simulink library "rappid_564xl_ec_toolbox"  (R2016b)
settings: Solver=FixedStepDiscrete  StartTime=0.0  StopTime=10.0  RelTol=1e-3  EnableMultiTasking=on
undefined symbols (not defined in the file or in its folder): CTU_unit, mem_AddrLW, mem_AddrUP, rappid_564xl_adc_input_support_rev2, rappid_564xl_can_support_rev2, read_mem_AddrLW, read_mem_AddrUP
(part 4 of 6)

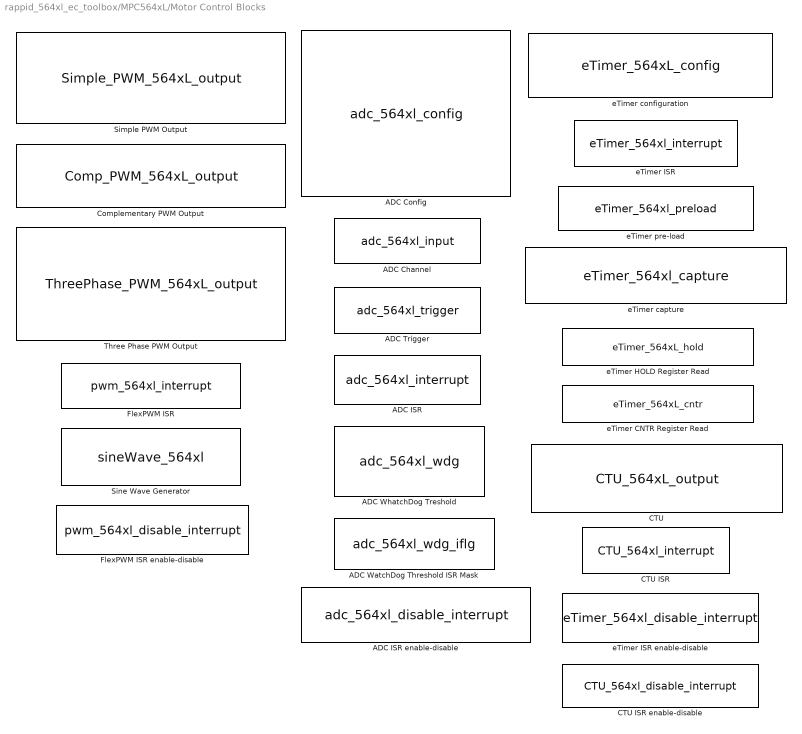
== system rappid_564xl_ec_toolbox/MPC564xL/Motor Control Blocks ==
  ADC Channel : S-Function  LoadFcn=rappid_564xl_adc_input_support_rev2(gcb)  FunctionName=adc_564xl_input  Parameters="adcChan, adc_unit, adc_mode, simulate,  interrupt, adc_presample"  SFunctionDeploymentMode=off  EnableBusSupport=off  mask(adc_564xl_input_block){adc_unit=1, adc_chan0=older, adc_chan0_v2=69 : PE5 : [44] : [T5] : AN8, adc_chan1=older, adc_chan1_v2=26 : PB10 : [53] : [R8] : AN12, simulate=off, interrupt=off, adc_mode=Normal, adc_presample=off}
      mask prompts: adc_unit "ADC Converter (0 - 1)"; adc_chan0 "ADC Channel"; adc_chan0_v2 "ADC Channel"; adc_chan1 "ADC Channel"; adc_chan1_v2 "ADC Channel"; simulate "Enable for Simulation"; adc_mode "Mode"; adc_presample "Presampling"
      mask help: This block allows the user to get samples from the ADC converter. The ADC is in a free run mode so all ADC samples are the latest in the ADC conversion register.
      mask init:
      | crlf = sprintf('\n');
      | 
      | adcInfoOut = rappid_564xl_adc_get_info(gcb);
      | 
      | adcChan = adcInfoOut.ChNum;
      | adcUnit = num2str(adcInfoOut.UnitNum);
      | adcMode = adcInfoOut.Mode;
      | maskStr = [ 'ADC Converter: ',adcUnit, crlf, 'ADC Channel: ',num2str(adcInfoOut.ChNum), crlf, 'ADC Mode: ', adcMode]; 
      | 
      | rappid_564xl_adc_input_support_rev2(gcb);
      | set_param(gcb, 'adc_chan0', 'older');
      | set_param(gcb, 'adc_chan1', 'older');
      mask Help: web([rappid_block_help,filesep,'adc_input_block.htm']);
      mask TypeOptions adc_unit: 0 | 1
      mask Callback adc_unit:
      | param = str2num(get_param ( gcb, 'adc_unit'));
      | MaskVis = get_param(gcb, 'MaskVisibilities');
      | 
      | if (param == 0)
      | 	MaskVis{2} = 'off';
      |     MaskVis{3} = 'on';
      |     MaskVis{4} = 'off';
      | 	MaskVis{5} = 'off';
      | elseif (param == 1)
      | 	MaskVis{2} = 'off';
      |     MaskVis{3} = 'off';
      |     MaskVis{4} = 'off';
      | 	MaskVis{5} = 'on';
      | end
      | 
      | set_param(gcb, 'MaskVisibilities', MaskVis);
      mask TypeOptions adc_chan0: PCR[23] : B[7] : 43 : R5 : AN[0] | PCR[24] : B[8] : 47 : P7 : AN[1] | PCR[25] : B[9] : 52 : U7 : AN[11] | PCR[26] : B[10] : 53: R8 : AN[12] | PCR[27] : B[11] : 54 : T8 : AN[13] | PCR[28] : B[12] : 55 : U8 : AN[14] | PCR[33] : C[1] : 41 : T4 : AN[2] | PCR[34] : C[2] : 45 : U5 : AN[3] | PCR[66] : E[2] : 49 : U6 : AN[5] | PCR[68] : E[4] : 42 : U4 : AN[7] | PCR[69] : E[5] : 44 : T5 : AN[8] | PCR[70] : E[6] : 46 : R6 : AN[4] | PCR[71] : E[7] : 48 : T6 : AN[6] | PCR[---] : [---] : [---] : [---] : AN[9] | PCR[---] : [---] : [---] : [---] : AN[10] | PCR[---] : [---] : [---] : [---] : AN[15] | older
      mask TypeOptions adc_chan0_v2: 23 : PB7 : [43] : [R5] : AN0 | 24 : PB8 : [47] : [P7] : AN1 | 25 : PB9 : [52] : [U7] : AN11 | 26 : PB10 : [53]: [R8] : AN12 | 27 : PB11 : [54] : [T8] : AN13 | 28 : PB12 : [55] : [U8] : AN14 | 33 : PC1 : [41] : [T4] : AN2 | 34 : PC2 : [45] : [U5] : AN3 | 66 : PE2 : [49] : [U6] : AN5 | 68 : PE4 : [42] : [U4] : AN7 | 69 : PE5 : [44] : [T5] : AN8 | 70 : PE6 : [46] : [R6] : AN4 | 71 : PE7 : [48] : [T6] : AN6 | --- : --- : [---] : [---] : AN9 | --- : --- : [---] : [---] : AN10 | --- : --- : [---] : [---] : AN15
      mask TypeOptions adc_chan1: PCR[25] : B[9] : 52 : U7 : AN[11] | PCR[26] : B10] : 53 : R8 : AN[12] | PCR[27] : B[11] : 54 : T8 : AN[13] | PCR[28] : B[12] : 55 : U8 : AN[14] | PCR[29] : B[13] : 60 : R10 : AN[0] | PCR[30] : B[14] : 64 : P11 : AN[1] | PCR[31] : B[15] : 62 : R11 : AN[2] | PCR[32] : C[0] : 66 : R12 : AN[3] | PCR[64] : E[0] : 68 : T13 : AN[5] | PCR[73] : E[9] : 61 : T10 : AN[7] | PCR[74] : E[10] : 63 : T11 : AN[8] | PCR[75] : E[11] : 65 : U11 : AN[4] | PCR[76] : E[12] : 67 : T12 : AN[6] | PCR[---] : [---] : [---] : [---] : AN[9] | PCR[---] : [---] : [---] : [---] : AN[10] | PCR[---] : [---] : [---] : [---] : AN[15] | older
      mask TypeOptions adc_chan1_v2: 25 : PB9 : [52] : [U7] : AN11 | 26 : PB10 : [53] : [R8] : AN12 | 27 : PB11 : [54] : [T8] : AN13 | 28 : PB12 : [55] : [U8] : AN14 | 29 : PB13 : [60] : [R10] : AN0 | 30 : PB14 : [64] : [P11] : AN1 | 31 : PB15 : [62] : [R11] : AN2 | 32 : PC0 : [66] : [R12] : AN3 | 64 : PE0 : [68] : [T13] : AN5 | 73 : PE9 : [61] : [T10] : AN7 | 74 : PE10 : [63] : [T11] : AN8 | 75 : PE11 : [65] : [U11] : AN4 | 76 : PE12 : [67] : [T12] : AN6 | --- : --- : [---] : [---] : AN9 | --- : --- : [---] : [---] : AN10 | --- : --- : [---] : [---] : AN15
      mask TypeOptions adc_mode: Normal | Injected
      mask Display: disp(maskStr)
  ADC Config : S-Function  FunctionName=adc_564xl_config  Parameters="adc_unit, adc_ctu, adc_owr, adc_wls, adc_clk, adc_ack, adc_ctr0_inp, adc_ctr0_shft, adc_ctr0_cmp, adc_ctr0_samp, adc_ctr1_inp,  adc_ctr1_cmp, adc_ctr1_samp, adcTSENS, adcPreVal0, adc_pscr_preconv"  SFunctionDeploymentMode=off  EnableBusSupport=off  mask(adc_564xl_config_block){adc_unit=0, adc_ctu=off, adc_owr=on, adc_wls=Left, adc_clk=on, adc_ack=on, adc_ctr0_inp=off, adc_ctr0_shft=10 - Avin = 0, adc_ctr0_cmp=01, adc_ctr0_samp=3, adc_ctr1_inp=off, adc_ctr1_cmp=01, adc_ctr1_samp=1, adc_ctr1_tsens=PTAT, adc_pscr_preval=V0, adc_pscr_preconv=off}
      mask prompts: adc_unit "ADC Converter (0 - 1)"; adc_ctu "CTU"; adc_owr "OWREN"; adc_wls "WLSIDE"; adc_clk "ADCLKSEL"; adc_ack "ACKO"; adc_ctr0_inp "INPLATCH"; adc_ctr0_shft "OFFSHIFT"; adc_ctr0_cmp "INPCMP"; adc_ctr0_samp "INPSAMP (3 - 255)"; adc_ctr1_inp "INPLATCH"; adc_ctr1_cmp "INPCMP"; adc_ctr1_samp "INPSAMP(1 - 127)"; adc_ctr1_tsens "TSENSOR_SEL"; adc_pscr_preval "PREVAL0"; adc_pscr_preconv "PRECONV"
      mask help: This block allows the user to configure ADC module.
      mask init:
      | crlf = sprintf('\n');
      | 
      | adcUnit = num2str(get_param(gcb,'adc_unit'));
      | adcCTU = num2str(get_param(gcb,'adc_ctu'));
      | adcOWR = num2str(get_param(gcb,'adc_owr'));
      | adcWLS = num2str(get_param(gcb,'adc_wls'));
      | adcCLK = num2str(get_param(gcb,'adc_clk'));
      | adcACK = num2str(get_param(gcb,'adc_ack'));
      | adcINP = num2str(get_param(gcb,'adc_ctr0_inp'));
      | adcSHFT= num2str(get_param(gcb,'adc_ctr0_shft'));
      | adcCMP = num2str(get_param(gcb,'adc_ctr0_cmp'));
      | adcSAMP= num2str(get_param(gcb,'adc_ctr0_samp'));
      | 
      | adcTSENS = get_param(gcb, 'adc_ctr1_tsens');
      | if (strcmp(adcTSENS, 'PTAT'))
      |     adcTSENS = 0;
      | else
      |     adcTSENS = 1;
      | end
      | 
      | adcPreVal0 = get_param(gcb, 'adc_pscr_preval');
      | if (strcmp(adcPreVal0,'V0'))
      |     adcPreVal0 = 0;
      | else
      |     adcPreVal0 = 1;
      | end
      | 
      | maskStr = [ 'ADC Converter ',adcUnit, crlf, 'ADC CTU mode ', adcCTU, crlf,...
      |     'Overwrite Enable ', adcOWR, crlf,'Left/Right write ',adcWLS, crlf,...
      |     'Analog Clock frequency selector ', adcCLK, crlf, 'Auto-clock-off ',...
      |     adcACK, crlf, 'Latching phase ', adcINP, crlf, 'Offset Shift ', adcSHFT,...
      |     crlf, 'Comparsion phase bits ', adcCMP, crlf, 'Sampling phase ', adcSAMP];
      mask Help: web([rappid_block_help,filesep,'adc_config_block.htm']);
      mask TypeOptions adc_unit: 0 | 1
      mask TypeOptions adc_wls: Left | Right
      mask TypeOptions adc_ctr0_shft: 00 - NoShift | 01 - Avin = 1/2LSB | 10 - Avin = 0
      mask TypeOptions adc_ctr0_cmp: 00 | 01 | 10 | 11
      mask Callback adc_ctr0_samp:
      | value = str2num(get_param(gcb, 'adc_ctr0_samp'));
      | if (value > 255)
      |     value = 255;
      | elseif (value < 3)
      |         value = 3;
      | end
      | set_param( gcb, 'adc_ctr0_samp', num2str(value));
      mask TypeOptions adc_ctr1_cmp: 00 | 01 | 10 | 11
      mask Callback adc_ctr1_samp:
      | value = str2num(get_param(gcb, 'adc_ctr1_samp'));
      | if (value > 127)
      |     value = 127;
      | elseif (value < 1)
      |         value = 1;
      | end
      | set_param( gcb, 'adc_ctr1_samp', num2str(value));
      mask TypeOptions adc_ctr1_tsens: PTAT | CTAT
      mask TypeOptions adc_pscr_preval: V0 | V1
      mask Display: disp(maskStr)
  ADC ISR : S-Function  FunctionName=adc_564xl_interrupt  Parameters=adc_unit, adc_isr_pri, adcIsrInfoOut  SFunctionDeploymentMode=off  EnableBusSupport=off  mask(adc_564xl_interrupt_block){adc_unit=0, adc_isr_pri=14, adc_isr_ech=off, adc_isr_eoc=off, adc_isr_jech=on, adc_isr_jeoc=on, adc_isr_eoctu=off}
      mask prompts: adc_unit "ADC Converter (0 - 1)"; adc_isr_pri "ISR priority (0 to 15)"; adc_isr_ech "ECH (End of the chain conversion)"; adc_isr_eoc "EOC (End of the channel conversion)"; adc_isr_jech "JECH (Injected end of the chain conversion)"; adc_isr_jeoc "JEOC (Injected end of the channel conversion)"; adc_isr_eoctu "EOCTU (End of CTU conversion)"
      mask help: This block allows call user function on ADC conversion event.
      mask init:
      | crlf = sprintf('\n');
      | [adcUnit, adcPri,adcIsrInfoOut]=rappid_564xl_adc_isr_get_param(gcb);
      | maskStr = [ 'ADC Converter ',num2str(adcUnit), crlf,'Priority ', num2str(adcPri)];
      mask Help: web([rappid_block_help,filesep,'adc_interrupt_block.htm']);
      mask TypeOptions adc_unit: 0 | 1
      mask TypeOptions adc_isr_pri: 0 | 1 | 2 | 3 | 4 | 5 | 6 | 7 | 8 | 9 | 10 | 11 | 12 | 13 | 14 | 15
      mask Display:
      | disp(maskStr)
      | port_label('output',1, 'function')
      | port_label('output',2, 'ISR Mask')
  ADC ISR enable-disable : S-Function  FunctionName=adc_564xl_disable_interrupt  Parameters=adcUnit, uint16(ISR_MASK), uint16(CH_MASK), uint32(WDG_MASK)  SFunctionDeploymentMode=off  EnableBusSupport=off  mask(adc_564xl_isr_disable){adc_unit=0, adc_eoctu=off, adc_jeoc=off, adc_jech=off, adc_eoc=off, adc_ech=off, adc_wdg_0=off, adc_wdg_1=off, adc_wdg_2=off, adc_wdg_3=off, adc_wdg_4=off, adc_wdg_5=off, adc_wdg_6=off, adc_wdg_7=off, adc_wdg_8=off, adc_wdg_9=off, adc_wdg_10=off, adc_wdg_11=off, adc_wdg_12=off, adc_wdg_13=off, adc_wdg_14=off, adc_wdg_15=off, adc_wdg_16=off, adc_wdg_17=off, adc_wdg_18=off, adc_wdg_19=off, adc_wdg_20=off, adc_wdg_21=off, adc_wdg_22=off, adc_wdg_23=off, adc_wdg_24=off, adc_wdg_25=off, adc_wdg_26=off, adc_wdg_27=off, adc_wdg_28=off, adc_wdg_29=off, adc_wdg_30=off, adc_wdg_31=off, adc_ch_0=off, adc_ch_1=off, adc_ch_2=off, adc_ch_3=off, adc_ch_4=off, adc_ch_5=off, adc_ch_6=off, adc_ch_7=off, adc_ch_8=off, adc_ch_9=off, adc_ch_10=off, adc_ch_11=off, adc_ch_12=off, adc_ch_13=off, adc_ch_14=off, adc_ch_15=off}
      mask prompts: adc_unit "ADC Converter (0 - 1)"; adc_eoctu "Enable EOCTU"; adc_jeoc "Enable JEOC"; adc_jech "Enable JECH"; adc_eoc "Enable EOC"; adc_ech "Enable ECH"; adc_wdg_0 "Enable WDG CH0 Low"; adc_wdg_1 "Enable WDG CH0 High"; adc_wdg_2 "Enable WDG CH1 Low"; adc_wdg_3 "Enable WDG CH1 High"; adc_wdg_4 "Enable WDG CH2 Low"; adc_wdg_5 "Enable WDG CH2 High"; adc_wdg_6 "Enable WDG CH3 Low"; adc_wdg_7 "Enable WDG CH3 High"; adc_wdg_8 "Enable WDG CH4 Low"; adc_wdg_9 "Enable WDG CH4 High"; adc_wdg_10 "Enable WDG CH5 Low"; adc_wdg_11 "Enable WDG CH5 High"; adc_wdg_12 "Enable WDG CH6 Low"; adc_wdg_13 "Enable WDG CH6 High"; adc_wdg_14 "Enable WDG CH7 Low"; adc_wdg_15 "Enable WDG CH7 High"; adc_wdg_16 "Enable WDG CH8 Low"; adc_wdg_17 "Enable WDG CH8 High"; adc_wdg_18 "Enable WDG CH9 Low"; adc_wdg_19 "Enable WDG CH9 High"; adc_wdg_20 "Enable WDG CH10 Low"; adc_wdg_21 "Enable WDG CH10 High"; adc_wdg_22 "Enable WDG CH11 Low"; adc_wdg_23 "Enable WDG CH11 High"; adc_wdg_24 "Enable WDG CH12 Low"; adc_wdg_25 "Enable WDG CH12 High"; adc_wdg_26 "Enable WDG CH13 Low"; adc_wdg_27 "Enable WDG CH13 High"; adc_wdg_28 "Enable WDG CH14 Low"; adc_wdg_29 "Enable WDG CH14 High"; adc_wdg_30 "Enable WDG CH15 Low"; adc_wdg_31 "Enable WDG CH15 High"; adc_ch_0 "Enable CH0"; adc_ch_1 "Enable CH1"; adc_ch_2 "Enable CH2"; adc_ch_3 "Enable CH3"; adc_ch_4 "Enable CH4"; adc_ch_5 "Enable CH5"; adc_ch_6 "Enable CH6"; adc_ch_7 "Enable CH7"; adc_ch_8 "Enable CH8"; adc_ch_9 "Enable CH9"; adc_ch_10 "Enable CH10"; adc_ch_11 "Enable CH11"; adc_ch_12 "Enable CH12"; adc_ch_13 "Enable CH13"; adc_ch_14 "Enable CH14"; adc_ch_15 "Enable CH15"
      mask help: This block allows to enable/disable all ADC ISR's.
      mask init:
      | crlf = sprintf('\n');
      | 
      | adcUnit = str2num(get_param(gcb, 'adc_unit'));
      | 
      | 
      | 
      | ISR_MASK = 0;
      | if ( strcmp(get_param(gcb, 'adc_eoctu'), 'on'))
      |     ISR_MASK = bitset(uint16(ISR_MASK), 5);
      | end
      | 
      | if ( strcmp(get_param(gcb, 'adc_jeoc'), 'on'))
      |     ISR_MASK = bitset(uint16(ISR_MASK), 4);
      | end
      | 
      | if ( strcmp(get_param(gcb, 'adc_jech'), 'on'))
      |     ISR_MASK = bitset(uint16(ISR_MASK), 3);
      | end
      | 
      | if ( strcmp(get_param(gcb, 'adc_eoc'), 'on'))
      |     ISR_MASK = bitset(uint16(ISR_MASK), 2);
      | end
      | 
      | if ( strcmp(get_param(gcb, 'adc_ech'), 'on'))
      |     ISR_MASK = bitset(uint16(ISR_MASK), 1);
      | end
      | 
      | WDG_MASK = 0;
      | for index = 0:31
      |     str = [ 'adc_wdg_', num2str(index)];
      |     if (strcmp( get_param(gcb, str), 'on'))
      |         WDG_MASK = bitset(uint32(WDG_MASK), index+1);
      |     end
      | end
      | 
      | CH_MASK = 0;
      | for index = 0:15
      |     str = [ 'adc_ch_', num2str(index)];
      |     if (strcmp( get_param(gcb, str), 'on'))
      |         CH_MASK = bitset(uint32(CH_MASK), index+1);
      |     end
      | end
      | 
      | maskStr = [ 'ADC Converter: ',num2str(adcUnit), crlf,...
      |     'ADC ISR mask: ',dec2bin( ISR_MASK, 16), crlf,...
      |     'ADC Ch mask:  ',dec2bin(CH_MASK, 16), crlf,...
      |     'ADC WDG mask: ',dec2bin( WDG_MASK, 32)];
      mask Help: web([rappid_block_help,filesep,'ADC_isr_enable.htm']);
      mask TypeOptions adc_unit: 0 | 1
      mask Display: disp(maskStr)
  ADC Trigger : S-Function  FunctionName=adc_564xl_trigger  Parameters=adc_unit, adc_mode  SFunctionDeploymentMode=off  EnableBusSupport=off  mask(adc_564xl_trigger_block){adc_unit=0, adc_mode=Normal}
      mask prompts: adc_unit "ADC Converter (0 - 1)"; adc_mode "Mode"
      mask help: This block allows get measure in One Shot or Injected Mode. The ADC moved from Free Scan to One Shot/Injected mode get conversion and return it back.
      mask init:
      | crlf = sprintf('\n');
      | 
      | adcUnit = num2str(get_param(gcb,'adc_unit'));
      | adcMode = num2str(get_param(gcb,'adc_mode'));
      | maskStr = [ 'ADC Converter ',adcUnit, crlf, 'ADC Mode ',adcMode];
      mask Help: web([rappid_block_help,filesep,'adc_trigger_block.htm']);
      mask TypeOptions adc_unit: 0 | 1
      mask TypeOptions adc_mode: Normal | Injected
      mask Display: disp(maskStr)
  ADC WatchDog Threshold ISR Mask : S-Function  LoadFcn=rappid_564xl_adc_input_support_rev2(gcb)  FunctionName=adc_564xl_wdg_iflg  Parameters=adcWdgOut  SFunctionDeploymentMode=off  EnableBusSupport=off  mask(adc_564xl_input_treshhold_iflg_block){adc_unit=0, adc_chan0=older, adc_chan0_v2=23 : PB7 : [43] : [R5] : AN0, adc_chan1=older, adc_chan1_v2=25 : PB9 : [52] : [U7] : AN11, adc_isr_mask=Low & High Value Mask - On}
      mask prompts: adc_unit "ADC Converter (0 - 1)"; adc_chan0 "ADC Channel"; adc_chan0_v2 "ADC Channel"; adc_chan1 "ADC Channel"; adc_chan1_v2 "ADC Channel"; adc_isr_mask "ISR Mask"
      mask help: This block allows to enable/disable ADC Watchdog Threshold ISR.
      mask init:
      | crlf = sprintf('\n');
      | 
      | adcWdgStruct = rappid_564xl_adc_wdg_iflg_get_info(gcb);
      | 
      | adcChan = num2str(adcWdgStruct.ChNum);
      | adcUnit = num2str(adcWdgStruct.UnitNum);
      | 
      | adcIsrMask = get_param(gcb, 'adc_isr_mask');
      | 
      | maskStr = [ 'ADC Converter: ',adcUnit, crlf,...
      |     'ADC Channel: ',adcChan, crlf,...
      |     adcIsrMask]; 
      | adcWdgOut = [adcWdgStruct.UnitNum, adcWdgStruct.ChNum, adcWdgStruct.adcIFlgValue];
      | 
      | %disable older PCR-value
      | rappid_564xl_adc_input_support_rev2(gcb);
      | set_param(gcb, 'adc_chan0', 'older');
      | set_param(gcb, 'adc_chan1', 'older');
      mask Help: web([rappid_block_help,filesep,'ADC_treshold_isr_en.htm']);
      mask TypeOptions adc_unit: 0 | 1
      mask Callback adc_unit:
      | param = str2num(get_param ( gcb, 'adc_unit'));
      | MaskVis = get_param(gcb, 'MaskVisibilities');
      | 
      | if (param == 0)
      | 	MaskVis{2} = 'off';
      |     MaskVis{3} = 'on';
      |     MaskVis{4} = 'off';
      | 	MaskVis{5} = 'off';
      | elseif (param == 1)
      | 	MaskVis{2} = 'off';
      |     MaskVis{3} = 'off';
      |     MaskVis{4} = 'off';
      | 	MaskVis{5} = 'on';
      | end
      | 
      | set_param(gcb, 'MaskVisibilities', MaskVis);
      mask TypeOptions adc_chan0: PCR[23] : B[7] : 43 : R5 : AN[0] | PCR[24] : B[8] : 47 : P7 : AN[1] | PCR[25] : B[9] : 52 : U7 : AN[11] | PCR[26] : B[10] : 53: R8 : AN[12] | PCR[27] : B[11] : 54 : T8 : AN[13] | PCR[28] : B[12] : 55 : U8 : AN[14] | PCR[33] : C[1] : 41 : T4 : AN[2] | PCR[34] : C[2] : 45 : U5 : AN[3] | PCR[66] : E[2] : 49 : U6 : AN[5] | PCR[68] : E[4] : 42 : U4 : AN[7] | PCR[69] : E[5] : 44 : T5 : AN[8] | PCR[70] : E[6] : 46 : R6 : AN[4] | PCR[71] : E[7] : 48 : T6 : AN[6] | PCR[---] : [---] : [---] : [---] : AN[9] | PCR[---] : [---] : [---] : [---] : AN[10] | PCR[---] : [---] : [---] : [---] : AN[15] | older
      mask TypeOptions adc_chan0_v2: 23 : PB7 : [43] : [R5] : AN0 | 24 : PB8 : [47] : [P7] : AN1 | 25 : PB9 : [52] : [U7] : AN11 | 26 : PB10 : [53]: [R8] : AN12 | 27 : PB11 : [54] : [T8] : AN13 | 28 : PB12 : [55] : [U8] : AN14 | 33 : PC1 : [41] : [T4] : AN2 | 34 : PC2 : [45] : [U5] : AN3 | 66 : PE2 : [49] : [U6] : AN5 | 68 : PE4 : [42] : [U4] : AN7 | 69 : PE5 : [44] : [T5] : AN8 | 70 : PE6 : [46] : [R6] : AN4 | 71 : PE7 : [48] : [T6] : AN6 | --- : --- : [---] : [---] : AN9 | --- : --- : [---] : [---] : AN10 | --- : --- : [---] : [---] : AN15
      mask TypeOptions adc_chan1: PCR[25] : B[9] : 52 : U7 : AN[11] | PCR[26] : B10] : 53 : R8 : AN[12] | PCR[27] : B[11] : 54 : T8 : AN[13] | PCR[28] : B[12] : 55 : U8 : AN[14] | PCR[29] : B[13] : 60 : R10 : AN[0] | PCR[30] : B[14] : 64 : P11 : AN[1] | PCR[31] : B[15] : 62 : R11 : AN[2] | PCR[32] : C[0] : 66 : R12 : AN[3] | PCR[64] : E[0] : 68 : T13 : AN[5] | PCR[73] : E[9] : 61 : T10 : AN[7] | PCR[74] : E[10] : 63 : T11 : AN[8] | PCR[75] : E[11] : 65 : U11 : AN[4] | PCR[76] : E[12] : 67 : T12 : AN[6] | PCR[---] : [---] : [---] : [---] : AN[9] | PCR[---] : [---] : [---] : [---] : AN[10] | PCR[---] : [---] : [---] : [---] : AN[15] | older
      mask TypeOptions adc_chan1_v2: 25 : PB9 : [52] : [U7] : AN11 | 26 : PB10 : [53] : [R8] : AN12 | 27 : PB11 : [54] : [T8] : AN13 | 28 : PB12 : [55] : [U8] : AN14 | 29 : PB13 : [60] : [R10] : AN0 | 30 : PB14 : [64] : [P11] : AN1 | 31 : PB15 : [62] : [R11] : AN2 | 32 : PC0 : [66] : [R12] : AN3 | 64 : PE0 : [68] : [T13] : AN5 | 73 : PE9 : [61] : [T10] : AN7 | 74 : PE10 : [63] : [T11] : AN8 | 75 : PE11 : [65] : [U11] : AN4 | 76 : PE12 : [67] : [T12] : AN6 | --- : --- : [---] : [---] : AN9 | --- : --- : [---] : [---] : AN10 | --- : --- : [---] : [---] : AN15
      mask TypeOptions adc_isr_mask: Low Value Mask - On | Low Value Mask - Off | High Value Mask - On | High Value Mask - Off | Low & High Value Mask - On | Low & High Value Mask - Off
      mask Display: disp(maskStr)
  ADC WhatchDog Treshold : S-Function  LoadFcn=rappid_564xl_adc_input_support_rev2(gcb)  FunctionName=adc_564xl_wdg  Parameters=adcWdgOut  SFunctionDeploymentMode=off  EnableBusSupport=off  mask(adc_564xl_input_treshhold_block){adc_unit=0, adc_chan0=older, adc_chan0_v2=23 : PB7 : [43] : [R5] : AN0, adc_chan1=older, adc_chan1_v2=25 : PB9 : [52] : [U7] : AN11, adc_treshold=Oops, adc_treshold_value=2000, adc_up_value=4095, adc_mask_up=on, adc_low_value=800, adc_mask_low=on, adc_isr_pri=12}
      mask prompts: adc_unit "ADC Converter (0 - 1)"; adc_chan0 "ADC Channel"; adc_chan0_v2 "ADC Channel"; adc_chan1 "ADC Channel"; adc_chan1_v2 "ADC Channel"; adc_treshold "Old Treshold"; adc_treshold_value "Old Value"; adc_up_value "Upper Value"; adc_mask_up "Upper ISR Mask"; adc_low_value "Lower Value"; adc_mask_low "Lower ISR Mask"; adc_isr_pri "ISR Priority (0-15)"
      mask help: This block allow continue hardware monitoring. When watchdog is set it monitors ADC channel and call user function if get value more/less than threshold value.
      mask init:
      | crlf = sprintf('\n');
      | 
      | adcWdgStruct = rappid_564xl_adc_wdg_get_info(gcb);
      | 
      | adcChan = num2str(adcWdgStruct.ChNum);
      | adcUnit = num2str(adcWdgStruct.UnitNum);
      | adcUpValue = num2str(adcWdgStruct.UpValue);
      | adcLowValue = num2str(adcWdgStruct.LowValue);
      | adcMaskUp = adcWdgStruct.maskUpTxt;
      | adcMaskLow = adcWdgStruct.maskLowTxt;
      | 
      | 
      | maskStr = [ 'ADC Converter: ',adcUnit, crlf,...
      |     'ADC Channel: ',adcChan, crlf,...
      |     'Up Value: ', adcUpValue, crlf,...
      |     'Up ISR Mask: ', adcMaskUp, crlf,...
      |     'Low Value: ', adcLowValue, crlf,...
      |     'Low ISR Mask: ', adcMaskLow]; 
      | 
      | adcWdgOut = [adcWdgStruct.UnitNum, adcWdgStruct.ChNum,...
      |     adcWdgStruct.UpValue, adcWdgStruct.LowValue, adcWdgStruct.maskUp,...
      |     adcWdgStruct.maskLow];
      | 
      | %disable older PCR-value
      | rappid_564xl_adc_input_support_rev2(gcb);
      | set_param(gcb, 'adc_chan0', 'older');
      | set_param(gcb, 'adc_chan1', 'older');
      mask Help: web([rappid_block_help,filesep,'adc_input_treshold_block.htm']);
      mask TypeOptions adc_unit: 0 | 1
      mask Callback adc_unit:
      | param = str2num(get_param ( gcb, 'adc_unit'));
      | MaskVis = get_param(gcb, 'MaskVisibilities');
      | 
      | if (param == 0)
      | 	MaskVis{2} = 'off';
      |     MaskVis{3} = 'on';
      |     MaskVis{4} = 'off';
      | 	MaskVis{5} = 'off';
      | elseif (param == 1)
      | 	MaskVis{2} = 'off';
      |     MaskVis{3} = 'off';
      |     MaskVis{4} = 'off';
      | 	MaskVis{5} = 'on';
      | end
      | 
      | set_param(gcb, 'MaskVisibilities', MaskVis);
      mask TypeOptions adc_chan0: PCR[23] : B[7] : 43 : R5 : AN[0] | PCR[24] : B[8] : 47 : P7 : AN[1] | PCR[25] : B[9] : 52 : U7 : AN[11] | PCR[26] : B[10] : 53: R8 : AN[12] | PCR[27] : B[11] : 54 : T8 : AN[13] | PCR[28] : B[12] : 55 : U8 : AN[14] | PCR[33] : C[1] : 41 : T4 : AN[2] | PCR[34] : C[2] : 45 : U5 : AN[3] | PCR[66] : E[2] : 49 : U6 : AN[5] | PCR[68] : E[4] : 42 : U4 : AN[7] | PCR[69] : E[5] : 44 : T5 : AN[8] | PCR[70] : E[6] : 46 : R6 : AN[4] | PCR[71] : E[7] : 48 : T6 : AN[6] | PCR[---] : [---] : [---] : [---] : AN[9] | PCR[---] : [---] : [---] : [---] : AN[10] | PCR[---] : [---] : [---] : [---] : AN[15] | older
      mask TypeOptions adc_chan0_v2: 23 : PB7 : [43] : [R5] : AN0 | 24 : PB8 : [47] : [P7] : AN1 | 25 : PB9 : [52] : [U7] : AN11 | 26 : PB10 : [53]: [R8] : AN12 | 27 : PB11 : [54] : [T8] : AN13 | 28 : PB12 : [55] : [U8] : AN14 | 33 : PC1 : [41] : [T4] : AN2 | 34 : PC2 : [45] : [U5] : AN3 | 66 : PE2 : [49] : [U6] : AN5 | 68 : PE4 : [42] : [U4] : AN7 | 69 : PE5 : [44] : [T5] : AN8 | 70 : PE6 : [46] : [R6] : AN4 | 71 : PE7 : [48] : [T6] : AN6 | --- : --- : [---] : [---] : AN9 | --- : --- : [---] : [---] : AN10 | --- : --- : [---] : [---] : AN15
      mask TypeOptions adc_chan1: PCR[25] : B[9] : 52 : U7 : AN[11] | PCR[26] : B10] : 53 : R8 : AN[12] | PCR[27] : B[11] : 54 : T8 : AN[13] | PCR[28] : B[12] : 55 : U8 : AN[14] | PCR[29] : B[13] : 60 : R10 : AN[0] | PCR[30] : B[14] : 64 : P11 : AN[1] | PCR[31] : B[15] : 62 : R11 : AN[2] | PCR[32] : C[0] : 66 : R12 : AN[3] | PCR[64] : E[0] : 68 : T13 : AN[5] | PCR[73] : E[9] : 61 : T10 : AN[7] | PCR[74] : E[10] : 63 : T11 : AN[8] | PCR[75] : E[11] : 65 : U11 : AN[4] | PCR[76] : E[12] : 67 : T12 : AN[6] | PCR[---] : [---] : [---] : [---] : AN[9] | PCR[---] : [---] : [---] : [---] : AN[10] | PCR[---] : [---] : [---] : [---] : AN[15] | older
      mask TypeOptions adc_chan1_v2: 25 : PB9 : [52] : [U7] : AN11 | 26 : PB10 : [53] : [R8] : AN12 | 27 : PB11 : [54] : [T8] : AN13 | 28 : PB12 : [55] : [U8] : AN14 | 29 : PB13 : [60] : [R10] : AN0 | 30 : PB14 : [64] : [P11] : AN1 | 31 : PB15 : [62] : [R11] : AN2 | 32 : PC0 : [66] : [R12] : AN3 | 64 : PE0 : [68] : [T13] : AN5 | 73 : PE9 : [61] : [T10] : AN7 | 74 : PE10 : [63] : [T11] : AN8 | 75 : PE11 : [65] : [U11] : AN4 | 76 : PE12 : [67] : [T12] : AN6 | --- : --- : [---] : [---] : AN9 | --- : --- : [---] : [---] : AN10 | --- : --- : [---] : [---] : AN15
      mask TypeOptions adc_treshold: Lower | Upper | Oops
      mask Callback adc_treshold:
      | mask = get_param(gcb, 'adc_treshold');
      | value = get_param(gcb, 'adc_treshold_value');
      | 
      | if ( 0 == strcmp(mask, 'Oops'))
      |     if (strcmp(mask,'Lower'))
      |         set_param(gcb,'adc_low_value', value);
      |         set_param(gcb,'adc_mask_low', 'on');
      |     elseif (strcmp(mask, 'Upper'))
      |         set_param(gcb,'adc_up_value', value);
      |         set_param(gcb,'adc_mask_up', 'on');
      |     end
      |     set_param(gcb, 'adc_treshold','Oops');
      | end
      mask TypeOptions adc_isr_pri: 0 | 1 | 2 | 3 | 4 | 5 | 6 | 7 | 8 | 9 | 10 | 11 | 12 | 13 | 14 | 15
      mask Display: disp(maskStr)
  CTU : S-Function  Priority=1  LoadFcn=|  InitFcn=CTU_unit = rappid_564xl_ctu_init();  FunctionName=CTU_564xL_output  Parameters=uint8(Mode),uint32(InputSelection),uint32(TriggerOutput_1),uint32(TriggerOutput_2),uint8(MRS),uint16(MaxDelay),CTU_unit.T_delay,uint32(ADC_CmdIndex_1),uint32(ADC_CmdIndex_2),CTU_unit.ADC_Cmd,uint8(extTgrPcr),uint8(extInPcr)  SFunctionDeploymentMode=off  EnableBusSupport=off  mask(CTU_564xL_output){ModeEdit=Triggered, Mode=0, MRSedit=PWM reload Rising edge, MRS=0, MaxDelay=0, ExtTgrPin_0=46  : PC14 : [ 103 ] : [ E15 ], ExtInPin_0=None, extTgrPcr=46, extInPcr=255, InputSelection=0, PWM_REL=Disabled, PWM_ODD_0=Disabled, PWM_ODD_1=Disabled, PWM_ODD_2=Disabled, PWM_ODD_3=Disabled, PWM_EVEN_0=Disabled, PWM_EVEN_1=Disabled, PWM_EVEN_2=Disabled, PWM_EVEN_3=Disabled, RPWM_0=Disabled, RPWM_1=Disabled, RPWM_2=Disabled, RPWM_3=Disabled, eTimer_0=Disabled, eTimer_1=Disabled, External=Disabled, TriggerOutput_1=0, TriggerOutput_2=0, ADC_CmdIndex_1=0, ADC_CmdIndex_2=0, ADC_Cmd_1=16384, ADC_Cmd_2=0, ADC_Cmd_3=0, ADC_Cmd_4=0, ADC_Cmd_5=0, ADC_Cmd_6=0, ADC_Cmd_7=0, ADC_Cmd_8=0, ADC_Cmd_9=0, ADC_Cmd_10=0, ADC_Cmd_11=0, ADC_Cmd_12=0, ADC_Cmd_13=0, ADC_Cmd_14=0, ADC_Cmd_15=0, ADC_Cmd_16=0, ADC_Cmd_17=0, ADC_Cmd_18=0, ADC_Cmd_19=0, ADC_Cmd_20=0, ADC_Cmd_21=0, ADC_Cmd_22=0, ADC_Cmd_23=0, ADC_Cmd_24=0, T0_E=off, T0_ETE=off, T0_T0E=off, T0_T1E=off, T0_T2E=off, T0_ADCE=off, T0_Delay=0, T1_E=off, T1_ETE=off, T1_T0E=off, T1_T1E=off, T1_T2E=off, T1_ADCE=off, T1_Delay=0, T2_E=off, T2_ETE=off, T2_T0E=off, T2_T1E=off, T2_T2E=off, T2_ADCE=off, T2_Delay=0, T3_E=off, T3_ETE=off, T3_T0E=off, T3_T1E=off, T3_T2E=off, T3_ADCE=off, T3_Delay=0, T4_E=off, T4_ETE=off, T4_T0E=off, T4_T1E=off, T4_T2E=off, T4_ADCE=off, T4_Delay=0, T5_E=off, T5_ETE=off, T5_T0E=off, T5_T1E=off, T5_T2E=off, T5_ADCE=off, T5_Delay=0, T6_E=off, T6_ETE=off, T6_T0E=off, T6_T1E=off, T6_T2E=off, T6_ADCE=off, T6_Delay=0, T7_E=off, T7_ETE=off, T7_T0E=off, T7_T1E=off, T7_T2E=off, T7_ADCE=off, T7_Delay=0, T_delay=0, ADC_Cmd=0, T0_ADC_num=0, T0_ADC_nlist=no commands, T1_ADC_num=0, T1_ADC_nlist=no commands, T2_ADC_num=0, T2_ADC_nlist=no commands, T3_ADC_num=0, T3_ADC_nlist=no commands, T4_ADC_num=0, T4_ADC_nlist=no commands, T5_ADC_num=0, T5_ADC_nlist=no commands, T6_ADC_num=0, T6_ADC_nlist=no commands, T7_ADC_num=0, T7_ADC_nlist=no commands, ADC_CMS_1=Single-conversion mode: ADC unit A, ADC_CIR_1=Disabled, ADC_FIFO_1=0, ADC_CHA_1=0, ADC_CHB_1=0, ADC_CMS_2=Single-conversion mode: ADC unit A, ADC_CIR_2=Disabled, ADC_FIFO_2=0, ADC_CHA_2=0, ADC_CHB_2=0, ADC_CMS_3=Single-conversion mode: ADC unit A, ADC_CIR_3=Disabled, ADC_FIFO_3=0, ADC_CHA_3=0, ADC_CHB_3=0, ADC_CMS_4=Single-conversion mode: ADC unit A, ADC_CIR_4=Disabled, ADC_FIFO_4=0, ADC_CHA_4=0, ADC_CHB_4=0, ADC_CMS_5=Single-conversion mode: ADC unit A, ADC_CIR_5=Disabled, ADC_FIFO_5=0, ADC_CHA_5=0, ADC_CHB_5=0, ADC_CMS_6=Single-conversion mode: ADC unit A, ADC_CIR_6=Disabled, ADC_FIFO_6=0, ADC_CHA_6=0, ADC_CHB_6=0, ADC_CMS_7=Single-conversion mode: ADC unit A, ADC_CIR_7=Disabled, ADC_FIFO_7=0, ADC_CHA_7=0, ADC_CHB_7=0, ADC_CMS_8=Single-conversion mode: ADC unit A, ADC_CIR_8=Disabled, ADC_FIFO_8=0, ADC_CHA_8=0, ADC_CHB_8=0, ADC_CMS_9=Single-conversion mode: ADC unit A, ADC_CIR_9=Disabled, ADC_FIFO_9=0, ADC_CHA_9=0, ADC_CHB_9=0, ADC_CMS_10=Single-conversion mode: ADC unit A, ADC_CIR_10=Disabled, ADC_FIFO_10=0, ADC_CHA_10=0, ADC_CHB_10=0, ADC_CMS_11=Single-conversion mode: ADC unit A, ADC_CIR_11=Disabled, ADC_FIFO_11=0, ADC_CHA_11=0, ADC_CHB_11=0, ADC_CMS_12=Single-conversion mode: ADC unit A, ADC_CIR_12=Disabled, ADC_FIFO_12=0, ADC_CHA_12=0, ADC_CHB_12=0, ADC_CMS_13=Single-conversion mode: ADC unit A, ADC_CIR_13=Disabled, ADC_FIFO_13=0, ADC_CHA_13=0, ADC_CHB_13=0, ADC_CMS_14=Single-conversion mode: ADC unit A, ADC_CIR_14=Disabled, ADC_FIFO_14=0, ADC_CHA_14=0, ADC_CHB_14=0, ADC_CMS_15=Single-conversion mode: ADC unit A, ADC_CIR_15=Disabled, ADC_FIFO_15=0, ADC_CHA_15=0, ADC_CHB_15=0, ADC_CMS_16=Single-conversion mode: ADC unit A, ADC_CIR_16=Disabled, ADC_FIFO_16=0, ADC_CHA_16=0, ADC_CHB_16=0, ADC_CMS_17=Single-conversion mode: ADC unit A, ADC_CIR_17=Disabled, ADC_FIFO_17=0, ADC_CHA_17=0, ADC_CHB_17=0, ADC_CMS_18=Single-conversion mode: ADC unit A, ADC_CIR_18=Disabled, ADC_FIFO_18=0, ADC_CHA_18=0, ADC_CHB_18=0, ADC_CMS_19=Single-conversion mode: ADC unit A, ADC_CIR_19=Disabled, ADC_FIFO_19=0, ADC_CHA_19=0, ADC_CHB_19=0, ADC_CMS_20=Single-conversion mode: ADC unit A, ADC_CIR_20=Disabled, ADC_FIFO_20=0, ADC_CHA_20=0, ADC_CHB_20=0, ADC_CMS_21=Single-conversion mode: ADC unit A, ADC_CIR_21=Disabled, ADC_FIFO_21=0, ADC_CHA_21=0, ADC_CHB_21=0, ADC_CMS_22=Single-conversion mode: ADC unit A, ADC_CIR_22=Disabled, ADC_FIFO_22=0, ADC_CHA_22=0, ADC_CHB_22=0, ADC_CMS_23=Single-conversion mode: ADC unit A, ADC_CIR_23=Disabled, ADC_FIFO_23=0, ADC_CHA_23=0, ADC_CHB_23=0, ADC_CMS_24=Single-conversion mode: ADC unit A, ADC_CIR_24=Disabled, ADC_FIFO_24=0, ADC_CHA_24=0, ADC_CHB_24=0, dst=|, T0_cmdNum=0, T0_ADC_CMS_1=Single-conversion mode: ADC unit A, T0_ADC_CIR_1=Disabled, T0_ADC_FIFO_1=0, T0_ADC_CHA_1=0, T0_ADC_CHB_1=0, T0_ADC_CMS_2=Single-conversion mode: ADC unit A, T0_ADC_CIR_2=Disabled, T0_ADC_FIFO_2=0, T0_ADC_CHA_2=0, T0_ADC_CHB_2=0, T0_ADC_CMS_3=Single-conversion mode: ADC unit A, T0_ADC_CIR_3=Disabled, T0_ADC_FIFO_3=0, T0_ADC_CHA_3=0, T0_ADC_CHB_3=0, T1_cmdNum=0, T1_ADC_CMS_1=Single-conversion mode: ADC unit A, T1_ADC_CIR_1=Disabled, T1_ADC_FIFO_1=0, T1_ADC_CHA_1=0, T1_ADC_CHB_1=0, T1_ADC_CMS_2=Single-conversion mode: ADC unit A, T1_ADC_CIR_2=Disabled, T1_ADC_FIFO_2=0, T1_ADC_CHA_2=0, T1_ADC_CHB_2=0, T1_ADC_CMS_3=Single-conversion mode: ADC unit A, T1_ADC_CIR_3=Disabled, T1_ADC_FIFO_3=0, T1_ADC_CHA_3=0, T1_ADC_CHB_3=0, ver=2}
      | CTU_unit = rappid_564xl_ctu_init_check();
      | CTU_unit.init();                   
      | disp_string = CTU_unit.display_st; 
      | set_param(gcb,'dst',disp_string);  
      | clear disp_string;
      mask dst=|
      | Triggered mode
      |       Input selection: 00000000 00000000 00000000 00000000
      | Trigger Output 0-3: 00000000 00000000 00000000 00000000
      | Trigger Output 4-7: 00000000 00000000 00000000 00000000
      | ADC command list size: 0
      mask prompts: ModeEdit "Trigger Generation mode"; Mode "Trigger Generation mode Data"; MRSedit "Master Reload Selection"; MRS "Master Reload Selection Data"; MaxDelay "Counter Stop Delay (mks)"; ExtTgrPin_0 "External trigger pin selection"; ExtInPin_0 "External input pin selection"; extTgrPcr "External trigger PCR"; extInPcr "External input PCR"; InputSelection "Input Selection Data"; PWM_REL "PWM reload"; PWM_ODD_0 "PWM channel 0 odd"; PWM_ODD_1 "PWM channel 1 odd"; PWM_ODD_2 "PWM channel 2 odd"; PWM_ODD_3 "PWM channel 3 odd"; PWM_EVEN_0 "PWM channel 0 even"; PWM_EVEN_1 "PWM channel 1 even"; PWM_EVEN_2 "PWM channel 2 even"; PWM_EVEN_3 "PWM channel 3 even"; RPWM_0 "Real PWM channel 0"; RPWM_1 "Real PWM channel 1"; RPWM_2 "Real PWM channel 2"; RPWM_3 "Real PWM channel 3"; eTimer_0 "eTimer 1"; eTimer_1 "eTimer 2"; TriggerOutput_1 "Trigger Output 1"; TriggerOutput_2 "Trigger Output 2"; ADC_CmdIndex_1 "ADC command index 1"; ADC_CmdIndex_2 "ADC command index 2"; ADC_Cmd_1 "ADC command 1"; ADC_Cmd_2 "ADC command 2"; ADC_Cmd_3 "ADC command 3"; ADC_Cmd_4 "ADC command 4"; ADC_Cmd_5 "ADC command 5"; ADC_Cmd_6 "ADC command 6"; ADC_Cmd_7 "ADC command 7"; ADC_Cmd_8 "ADC command 8"; ADC_Cmd_9 "ADC command 9"; ADC_Cmd_10 "ADC command 10"; ADC_Cmd_11 "ADC command 11"; ADC_Cmd_12 "ADC command 12"; ADC_Cmd_13 "ADC command 13"; ADC_Cmd_14 "ADC command 14"; ADC_Cmd_15 "ADC command 15"; ADC_Cmd_16 "ADC command 16"; ADC_Cmd_17 "ADC command 17"; ADC_Cmd_18 "ADC command 18"; ADC_Cmd_19 "ADC command 19"; ADC_Cmd_20 "ADC command 20"; ADC_Cmd_21 "ADC command 21"; ADC_Cmd_22 "ADC command 22"; ADC_Cmd_23 "ADC command 23"; ADC_Cmd_24 "ADC command 24"; T0_E "Trigger 0 enable"; T0_ETE "Trigger 0 External output enable"; T0_T0E "Trigger 0 Timer 0 output enable"; T0_T1E "Trigger 0 Timer 1 output enable"; T0_T2E "Trigger 0 Timer 2 output enable"; T0_ADCE "Trigger 0 ADC command enable"; T0_Delay "Trigger 0 Delay (mks)"; T1_E "Trigger 1 enable"; T1_ETE "Trigger 1 External output enable"; T1_T0E "Trigger 1 Timer 0 output enable"; T1_T1E "Trigger 1 Timer 1 output enable"; T1_T2E "Trigger 1 Timer 2 output enable"; T1_ADCE "Trigger 1 ADC command enable"; T1_Delay "Trigger 1 Delay (mks)"; T2_E "Trigger 2 enable"; T2_ETE "Trigger 2 External output enable"; T2_T0E "Trigger 2 Timer 0 output enable"; T2_T1E "Trigger 2 Timer 1 output enable"; T2_T2E "Trigger 2 Timer 2 output enable"; T2_ADCE "Trigger 2 ADC command enable"; T2_Delay "Trigger 2 Delay (mks)"; T3_E "Trigger 3 enable"; T3_ETE "Trigger 3 External output enable"; T3_T0E "Trigger 3 Timer 0 output enable"; T3_T1E "Trigger 3 Timer 1 output enable"; T3_T2E "Trigger 3 Timer 2 output enable"; T3_ADCE "Trigger 3 ADC command enable"; T3_Delay "Trigger 3 Delay (mks)"; T4_E "Trigger 4 enable"; T4_ETE "Trigger 4 External output enable"; T4_T0E "Trigger 4 Timer 0 output enable"; T4_T1E "Trigger 4 Timer 1 output enable"; T4_T2E "Trigger 4 Timer 2 output enable"; T4_ADCE "Trigger 4 ADC command enable"; T4_Delay "Trigger 4 Delay (mks)"; T5_E "Trigger 5 enable"; T5_ETE "Trigger 5 External output enable"; T5_T0E "Trigger 5 Timer 0 output enable"; T5_T1E "Trigger 5 Timer 1 output enable"; T5_T2E "Trigger 5 Timer 2 output enable"; T5_ADCE "Trigger 5 ADC command enable"; T5_Delay "Trigger 5 Delay (mks)"; T6_E "Trigger 6 enable"; T6_ETE "Trigger 6 External output enable"; T6_T0E "Trigger 6 Timer 0 output enable"; T6_T1E "Trigger 6 Timer 1 output enable"; T6_T2E "Trigger 6 Timer 2 output enable"; T6_ADCE "Trigger 6 ADC command enable"; T6_Delay "Trigger 6 Delay (mks)"; T7_E "Trigger 7 enable"; T7_ETE "Trigger 7 External output enable"; T7_T0E "Trigger 7 Timer 0 output enable"; T7_T1E "Trigger 7 Timer 1 output enable"; T7_T2E "Trigger 7 Timer 2 output enable"; T7_ADCE "Trigger 7 ADC command enable"; T7_Delay "Trigger 7 Delay (mks)"; T0_ADC_num "Trigger 0 ADC Commands number"; T0_ADC_nlist "Trigger 0 ADC Commands"; T1_ADC_num "Trigger 1 ADC Commands number"; T1_ADC_nlist "Trigger 1 ADC Commands"; T2_ADC_num "Trigger 2 ADC Commands number"; T2_ADC_nlist "Trigger 2 ADC Commands"; T3_ADC_num "Trigger 3 ADC Commands number"; T3_ADC_nlist "Trigger 3 ADC Commands"; T4_ADC_num "Trigger 4 ADC Commands number"; T4_ADC_nlist "Trigger 4 ADC Commands"; T5_ADC_num "Trigger 5 ADC Commands number"; T5_ADC_nlist "Trigger 5 ADC Commands"; T6_ADC_num "Trigger 6 ADC Commands number"; T6_ADC_nlist "Trigger 6 ADC Commands"; T7_ADC_num "Trigger 7 ADC Commands number"; T7_ADC_nlist "Trigger 7 ADC Commands"; ADC_CMS_1 "Command 1: Conversion mode selection"; ADC_CIR_1 "Command 1: Command Interrupt Request"; ADC_FIFO_1 "Command 1: FIFO for ADC unit A/B"; ADC_CHA_1 "Command 1: ADC unit A channel number"; ADC_CHB_1 "Command 1: ADC unit B channel number"; ADC_CMS_2 "Command 2: Conversion mode selection"; ADC_CIR_2 "Command 2: Command Interrupt Request"; ADC_FIFO_2 "Command 2: FIFO for ADC unit A/B"; ADC_CHA_2 "Command 2: ADC unit A channel number"; ADC_CHB_2 "Command 2: ADC unit B channel number"; ADC_CMS_3 "Command 3: Conversion mode selection"; ADC_CIR_3 "Command 3: Command Interrupt Request"; ADC_FIFO_3 "Command 3: FIFO for ADC unit A/B"; ADC_CHA_3 "Command 3: ADC unit A channel number"; ADC_CHB_3 "Command 3: ADC unit B channel number"; ADC_CMS_4 "Command 4: Conversion mode selection"; ADC_CIR_4 "Command 4: Command Interrupt Request"; ADC_FIFO_4 "Command 4: FIFO for ADC unit A/B"; ADC_CHA_4 "Command 4: ADC unit A channel number"; ADC_CHB_4 "Command 4: ADC unit B channel number"; ADC_CMS_5 "Command 5: Conversion mode selection"; ADC_CIR_5 "Command 5: Command Interrupt Request"; ADC_FIFO_5 "Command 5: FIFO for ADC unit A/B"; ADC_CHA_5 "Command 5: ADC unit A channel number"; ADC_CHB_5 "Command 5: ADC unit B channel number"; ADC_CMS_6 "Command 6: Conversion mode selection"; ADC_CIR_6 "Command 6: Command Interrupt Request"; ADC_FIFO_6 "Command 6: FIFO for ADC unit A/B"; ADC_CHA_6 "Command 6: ADC unit A channel number"; ADC_CHB_6 "Command 6: ADC unit B channel number"; ADC_CMS_7 "Command 7: Conversion mode selection"; ADC_CIR_7 "Command 7: Command Interrupt Request"; ADC_FIFO_7 "Command 7: FIFO for ADC unit A/B"; ADC_CHA_7 "Command 7: ADC unit A channel number"; ADC_CHB_7 "Command 7: ADC unit B channel number"; ADC_CMS_8 "Command 8: Conversion mode selection"; ADC_CIR_8 "Command 8: Command Interrupt Request"; ADC_FIFO_8 "Command 8: FIFO for ADC unit A/B"; ADC_CHA_8 "Command 8: ADC unit A channel number"; ADC_CHB_8 "Command 8: ADC unit B channel number"; ADC_CMS_9 "Command 9: Conversion mode selection"; ADC_CIR_9 "Command 9: Command Interrupt Request"; ADC_FIFO_9 "Command 9: FIFO for ADC unit A/B"; ADC_CHA_9 "Command 9: ADC unit A channel number"; ADC_CHB_9 "Command 9: ADC unit B channel number"; ADC_CMS_10 "Command 10: Conversion mode selection"; ADC_CIR_10 "Command 10: Command Interrupt Request"; ADC_FIFO_10 "Command 10: FIFO for ADC unit A/B"; ADC_CHA_10 "Command 10: ADC unit A channel number"; ADC_CHB_10 "Command 10: ADC unit B channel number"; ADC_CMS_11 "Command 11: Conversion mode selection"; ADC_CIR_11 "Command 11: Command Interrupt Request"; ADC_FIFO_11 "Command 11: FIFO for ADC unit A/B"; ADC_CHA_11 "Command 11: ADC unit A channel number"; ADC_CHB_11 "Command 11: ADC unit B channel number"; ADC_CMS_12 "Command 12: Conversion mode selection"; ADC_CIR_12 "Command 12: Command Interrupt Request"; ADC_FIFO_12 "Command 12: FIFO for ADC unit A/B"; ADC_CHA_12 "Command 12: ADC unit A channel number"; ADC_CHB_12 "Command 12: ADC unit B channel number"; ADC_CMS_13 "Command 13: Conversion mode selection"; ADC_CIR_13 "Command 13: Command Interrupt Request"; ADC_FIFO_13 "Command 13: FIFO for ADC unit A/B"; ADC_CHA_13 "Command 13: ADC unit A channel number"; ADC_CHB_13 "Command 13: ADC unit B channel number"; ADC_CMS_14 "Command 14: Conversion mode selection"; ADC_CIR_14 "Command 14: Command Interrupt Request"; ADC_FIFO_14 "Command 14: FIFO for ADC unit A/B"; ADC_CHA_14 "Command 14: ADC unit A channel number"; ADC_CHB_14 "Command 14: ADC unit B channel number"; ADC_CMS_15 "Command 15: Conversion mode selection"; ADC_CIR_15 "Command 15: Command Interrupt Request"; ADC_FIFO_15 "Command 15: FIFO for ADC unit A/B"; ADC_CHA_15 "Command 15: ADC unit A channel number"; ADC_CHB_15 "Command 15: ADC unit B channel number"; ADC_CMS_16 "Command 16: Conversion mode selection"; ADC_CIR_16 "Command 16: Command Interrupt Request"; ADC_FIFO_16 "Command 16: FIFO for ADC unit A/B"; ADC_CHA_16 "Command 16: ADC unit A channel number"; ADC_CHB_16 "Command 16: ADC unit B channel number"; ADC_CMS_17 "Command 17: Conversion mode selection"; ADC_CIR_17 "Command 17: Command Interrupt Request"; ADC_FIFO_17 "Command 17: FIFO for ADC unit A/B"; ADC_CHA_17 "Command 17: ADC unit A channel number"; ADC_CHB_17 "Command 17: ADC unit B channel number"; ADC_CMS_18 "Command 18: Conversion mode selection"; ADC_CIR_18 "Command 18: Command Interrupt Request"; ADC_FIFO_18 "Command 18: FIFO for ADC unit A/B"; ADC_CHA_18 "Command 18: ADC unit A channel number"; ADC_CHB_18 "Command 18: ADC unit B channel number"; ADC_CMS_19 "Command 19: Conversion mode selection"; ADC_CIR_19 "Command 19: Command Interrupt Request"; ADC_FIFO_19 "Command 19: FIFO for ADC unit A/B"; ADC_CHA_19 "Command 19: ADC unit A channel number"; ADC_CHB_19 "Command 19: ADC unit B channel number"; ADC_CMS_20 "Command 20: Conversion mode selection"; ADC_CIR_20 "Command 20: Command Interrupt Request"; ADC_FIFO_20 "Command 20: FIFO for ADC unit A/B"; ADC_CHA_20 "Command 20: ADC unit A channel number"; ADC_CHB_20 "Command 20: ADC unit B channel number"; ADC_CMS_21 "Command 21: Conversion mode selection"; ADC_CIR_21 "Command 21: Command Interrupt Request"; ADC_FIFO_21 "Command 21: FIFO for ADC unit A/B"; ADC_CHA_21 "Command 21: ADC unit A channel number"; ADC_CHB_21 "Command 21: ADC unit B channel number"; ADC_CMS_22 "Command 22: Conversion mode selection"; ADC_CIR_22 "Command 22: Command Interrupt Request"; ADC_FIFO_22 "Command 22: FIFO for ADC unit A/B"; ADC_CHA_22 "Command 22: ADC unit A channel number"; ADC_CHB_22 "Command 22: ADC unit B channel number"; ADC_CMS_23 "Command 23: Conversion mode selection"; ADC_CIR_23 "Command 23: Command Interrupt Request"; ADC_FIFO_23 "Command 23: FIFO for ADC unit A/B"; ADC_CHA_23 "Command 23: ADC unit A channel number"; ADC_CHB_23 "Command 23: ADC unit B channel number"; ADC_CMS_24 "Command 24: Conversion mode selection"; ADC_CIR_24 "Command 24: Command Interrupt Request"; ADC_FIFO_24 "Command 24: FIFO for ADC unit A/B"; ADC_CHA_24 "Command 24: ADC unit A channel number"; ADC_CHB_24 "Command 24: ADC unit B channel number"; dst "Dispaying string"; T0_cmdNum "depricated"; T0_ADC_CMS_1 "depricated"; T0_ADC_CIR_1 "depricated"; T0_ADC_FIFO_1 "depricated"; T0_ADC_CHA_1 "depricated"; T0_ADC_CHB_1 "depricated"; T0_ADC_CMS_2 "depricated"; T0_ADC_CIR_2 "depricated"; T0_ADC_FIFO_2 "depricated"; T0_ADC_CHA_2 "depricated"; T0_ADC_CHB_2 "depricated"; T0_ADC_CMS_3 "depricated"; T0_ADC_CIR_3 "depricated"; T0_ADC_FIFO_3 "depricated"; T0_ADC_CHA_3 "depricated"; T0_ADC_CHB_3 "depricated"; T1_cmdNum "depricated"; T1_ADC_CMS_1 "depricated"; T1_ADC_CIR_1 "depricated"; T1_ADC_FIFO_1 "depricated"; T1_ADC_CHA_1 "depricated"; T1_ADC_CHB_1 "depricated"; T1_ADC_CMS_2 "depricated"; T1_ADC_CIR_2 "depricated"; T1_ADC_FIFO_2 "depricated"; T1_ADC_CHA_2 "depricated"; T1_ADC_CHB_2 "depricated"; T1_ADC_CMS_3 "depricated"; T1_ADC_CIR_3 "depricated"; T1_ADC_FIFO_3 "depricated"; T1_ADC_CHA_3 "depricated"; T1_ADC_CHB_3 "depricated"; ver "version"
      mask help: Cross Triggering Unit block to configure CTU mode and its interfaces with other peripherals.
      mask init:
      | st = get_param(gcb,'dst');
      settings: CopyFcn=set_param(gcb,'ver','2');  DeleteFcn=rappid_564xl_ctu_clear();  ModelCloseFcn=rappid_564xl_ctu_clear();  PreCopyFcn=CTU_unit = rappid_564xl_ctu_init();  OpenFcn=set_param(gcb,'ver','2'); open_system(gcb,'mask');  MoveFcn=set_param(gcb,'ver','2');
      mask Help: web([rappid_block_help,filesep,'CTU_output.htm']);
      mask TypeOptions ModeEdit: Triggered | Sequential
      mask Callback ModeEdit:
      | maskParams = get_param(gcb,'MaskPrompts');
      | MaskEnables = get_param(gcb,'MaskEnables');
      | ModeEdit = get_param(gcb,'ModeEdit');
      | for i = 1:length(maskParams)
      |     if strcmp(maskParams{i},'Master Reload Selection')==1
      |         if strcmp(ModeEdit,'Triggered')==0
      |             MaskEnables{i} = 'on';
      |         else
      |             MaskEnables{i} = 'off';
      |         end
      |         break
      |     end
      | end
      | set_param(gcb,'MaskEnables',MaskEnables);
      mask TypeOptions MRSedit: PWM reload Rising edge | PWM reload Falling edge | PWM channel 0 odd Rising edge | PWM channel 0 odd Falling edge | PWM channel 1 odd Rising edge | PWM channel 1 odd Falling edge | PWM channel 2 odd Rising edge | PWM channel 2 odd Falling edge | PWM channel 3 odd Rising edge | PWM channel 3 odd Falling edge | PWM channel 0 even Rising edge | PWM channel 0 even Falling edge | PWM channel 1 even Rising edge | PWM channel 1 even Falling edge | PWM channel 2 even Rising edge | PWM channel 2 even Falling edge | PWM channel 3 even Rising edge | PWM channel 3 even Falling edge | Real PWM channel 0 Rising edge | Real PWM channel 0 Falling edge | Real PWM channel 1 Rising edge | Real PWM channel 1 Falling edge | Real PWM channel 2 Rising edge | Real PWM channel 2 Falling edge | Real PWM channel 3 Rising edge | Real PWM channel 3 Falling edge | eTimer 1 Rising edge | eTimer 1 Falling edge | eTimer 2 Rising edge | eTimer 2 Falling edge | External signal Rising edge | External signal Falling edge
      mask TypeOptions ExtTgrPin_0: None | 46  : PC14 : [ 103 ] : [ E15 ] | 49  : PD1  : [ 3 ] : [ E3 ] | 131 : PI3  : [ --- ] : [ E17 ]
      mask TypeOptions ExtInPin_0: None | 45  : PC13 : [ 101 ] : [ F15 ] | 47  : PC15 : [ 124 ] : [ A8 ]
      mask TypeOptions PWM_REL: Disabled | Rising | Falling | Rising and Falling
      mask TypeOptions PWM_ODD_0: Disabled | Rising | Falling | Rising and Falling
      mask TypeOptions PWM_ODD_1: Disabled | Rising | Falling | Rising and Falling
      mask TypeOptions PWM_ODD_2: Disabled | Rising | Falling | Rising and Falling
      mask TypeOptions PWM_ODD_3: Disabled | Rising | Falling | Rising and Falling
      mask TypeOptions PWM_EVEN_0: Disabled | Rising | Falling | Rising and Falling
      mask TypeOptions PWM_EVEN_1: Disabled | Rising | Falling | Rising and Falling
      mask TypeOptions PWM_EVEN_2: Disabled | Rising | Falling | Rising and Falling
      mask TypeOptions PWM_EVEN_3: Disabled | Rising | Falling | Rising and Falling
      mask TypeOptions RPWM_0: Disabled | Rising | Falling | Rising and Falling
      mask TypeOptions RPWM_1: Disabled | Rising | Falling | Rising and Falling
      mask TypeOptions RPWM_2: Disabled | Rising | Falling | Rising and Falling
      mask TypeOptions RPWM_3: Disabled | Rising | Falling | Rising and Falling
      mask TypeOptions eTimer_0: Disabled | Rising | Falling | Rising and Falling
      mask TypeOptions eTimer_1: Disabled | Rising | Falling | Rising and Falling
      mask TypeOptions External: Disabled | Rising | Falling | Rising and Falling
      mask Callback T0_E: CTU_unit.OnStateChange(0);
      mask Callback T0_ADCE: CTU_unit.ADC_OnStateChange(0);
      mask Callback T1_E: CTU_unit.OnStateChange(1);
      mask Callback T1_ADCE: CTU_unit.ADC_OnStateChange(1);
      mask Callback T2_E: CTU_unit.OnStateChange(2);
      mask Callback T2_ADCE: CTU_unit.ADC_OnStateChange(2);
      mask Callback T3_E: CTU_unit.OnStateChange(3);
      mask Callback T3_ADCE: CTU_unit.ADC_OnStateChange(3);
      mask Callback T4_E: CTU_unit.OnStateChange(4);
      mask Callback T4_ADCE: CTU_unit.ADC_OnStateChange(4);
      mask Callback T5_E: CTU_unit.OnStateChange(5);
      mask Callback T5_ADCE: CTU_unit.ADC_OnStateChange(5);
      mask Callback T6_E: CTU_unit.OnStateChange(6);
      mask Callback T6_ADCE: CTU_unit.ADC_OnStateChange(6);
      mask Callback T7_E: CTU_unit.OnStateChange(7);
      mask Callback T7_ADCE: CTU_unit.ADC_OnStateChange(7);
      mask TypeOptions T0_ADC_num: 0 | 1 | 2 | 3 | 4 | 5 | 6 | 7 | 8 | 9 | 10 | 11 | 12 | 13 | 14 | 15 | 16 | 17 | 18 | 19 | 20 | 21 | 22 | 23 | 24
      mask Callback T0_ADC_num: rappid_564xl_ctu_adc_cmd_num(gcb,0);
      mask TypeOptions T1_ADC_num: 0 | 1 | 2 | 3 | 4 | 5 | 6 | 7 | 8 | 9 | 10 | 11 | 12 | 13 | 14 | 15 | 16 | 17 | 18 | 19 | 20 | 21 | 22 | 23 | 24
      mask Callback T1_ADC_num: rappid_564xl_ctu_adc_cmd_num(gcb,1);
      mask TypeOptions T2_ADC_num: 0 | 1 | 2 | 3 | 4 | 5 | 6 | 7 | 8 | 9 | 10 | 11 | 12 | 13 | 14 | 15 | 16 | 17 | 18 | 19 | 20 | 21 | 22 | 23 | 24
      mask Callback T2_ADC_num: rappid_564xl_ctu_adc_cmd_num(gcb,2);
      mask TypeOptions T3_ADC_num: 0 | 1 | 2 | 3 | 4 | 5 | 6 | 7 | 8 | 9 | 10 | 11 | 12 | 13 | 14 | 15 | 16 | 17 | 18 | 19 | 20 | 21 | 22 | 23 | 24
      mask Callback T3_ADC_num: rappid_564xl_ctu_adc_cmd_num(gcb,3);
      mask TypeOptions T4_ADC_num: 0 | 1 | 2 | 3 | 4 | 5 | 6 | 7 | 8 | 9 | 10 | 11 | 12 | 13 | 14 | 15 | 16 | 17 | 18 | 19 | 20 | 21 | 22 | 23 | 24
      mask Callback T4_ADC_num: rappid_564xl_ctu_adc_cmd_num(gcb,4);
      mask TypeOptions T5_ADC_num: 0 | 1 | 2 | 3 | 4 | 5 | 6 | 7 | 8 | 9 | 10 | 11 | 12 | 13 | 14 | 15 | 16 | 17 | 18 | 19 | 20 | 21 | 22 | 23 | 24
      mask Callback T5_ADC_num: rappid_564xl_ctu_adc_cmd_num(gcb,5);
      mask TypeOptions T6_ADC_num: 0 | 1 | 2 | 3 | 4 | 5 | 6 | 7 | 8 | 9 | 10 | 11 | 12 | 13 | 14 | 15 | 16 | 17 | 18 | 19 | 20 | 21 | 22 | 23 | 24
      mask Callback T6_ADC_num: rappid_564xl_ctu_adc_cmd_num(gcb,6);
      mask TypeOptions T7_ADC_num: 0 | 1 | 2 | 3 | 4 | 5 | 6 | 7 | 8 | 9 | 10 | 11 | 12 | 13 | 14 | 15 | 16 | 17 | 18 | 19 | 20 | 21 | 22 | 23 | 24
      mask Callback T7_ADC_num: rappid_564xl_ctu_adc_cmd_num(gcb,7);
      mask TypeOptions ADC_CMS_1: Single-conversion mode: ADC unit A | Single-conversion mode: ADC unit B | Dual-conversion mode
      mask TypeOptions ADC_CIR_1: Disabled | Enabled
      mask TypeOptions ADC_FIFO_1: 0 | 1 | 2 | 3 | 4 | 5 | 6 | 7
      mask TypeOptions ADC_CHA_1: 0 | 1 | 2 | 3 | 4 | 5 | 6 | 7 | 8 | 9 | 10 | 11 | 12 | 13 | 14 | 15
      mask TypeOptions ADC_CHB_1: 0 | 1 | 2 | 3 | 4 | 5 | 6 | 7 | 8 | 9 | 10 | 11 | 12 | 13 | 14 | 15
      mask TypeOptions ADC_CMS_2: Single-conversion mode: ADC unit A | Single-conversion mode: ADC unit B | Dual-conversion mode
      mask TypeOptions ADC_CIR_2: Disabled | Enabled
      mask TypeOptions ADC_FIFO_2: 0 | 1 | 2 | 3 | 4 | 5 | 6 | 7
      mask TypeOptions ADC_CHA_2: 0 | 1 | 2 | 3 | 4 | 5 | 6 | 7 | 8 | 9 | 10 | 11 | 12 | 13 | 14 | 15
      mask TypeOptions ADC_CHB_2: 0 | 1 | 2 | 3 | 4 | 5 | 6 | 7 | 8 | 9 | 10 | 11 | 12 | 13 | 14 | 15
      mask TypeOptions ADC_CMS_3: Single-conversion mode: ADC unit A | Single-conversion mode: ADC unit B | Dual-conversion mode
      mask TypeOptions ADC_CIR_3: Disabled | Enabled
      mask TypeOptions ADC_FIFO_3: 0 | 1 | 2 | 3 | 4 | 5 | 6 | 7
      mask TypeOptions ADC_CHA_3: 0 | 1 | 2 | 3 | 4 | 5 | 6 | 7 | 8 | 9 | 10 | 11 | 12 | 13 | 14 | 15
      mask TypeOptions ADC_CHB_3: 0 | 1 | 2 | 3 | 4 | 5 | 6 | 7 | 8 | 9 | 10 | 11 | 12 | 13 | 14 | 15
      mask TypeOptions ADC_CMS_4: Single-conversion mode: ADC unit A | Single-conversion mode: ADC unit B | Dual-conversion mode
      mask TypeOptions ADC_CIR_4: Disabled | Enabled
      mask TypeOptions ADC_FIFO_4: 0 | 1 | 2 | 3 | 4 | 5 | 6 | 7
      mask TypeOptions ADC_CHA_4: 0 | 1 | 2 | 3 | 4 | 5 | 6 | 7 | 8 | 9 | 10 | 11 | 12 | 13 | 14 | 15
      mask TypeOptions ADC_CHB_4: 0 | 1 | 2 | 3 | 4 | 5 | 6 | 7 | 8 | 9 | 10 | 11 | 12 | 13 | 14 | 15
      mask TypeOptions ADC_CMS_5: Single-conversion mode: ADC unit A | Single-conversion mode: ADC unit B | Dual-conversion mode
      mask TypeOptions ADC_CIR_5: Disabled | Enabled
      mask TypeOptions ADC_FIFO_5: 0 | 1 | 2 | 3 | 4 | 5 | 6 | 7
      mask TypeOptions ADC_CHA_5: 0 | 1 | 2 | 3 | 4 | 5 | 6 | 7 | 8 | 9 | 10 | 11 | 12 | 13 | 14 | 15
      mask TypeOptions ADC_CHB_5: 0 | 1 | 2 | 3 | 4 | 5 | 6 | 7 | 8 | 9 | 10 | 11 | 12 | 13 | 14 | 15
      mask TypeOptions ADC_CMS_6: Single-conversion mode: ADC unit A | Single-conversion mode: ADC unit B | Dual-conversion mode
      mask TypeOptions ADC_CIR_6: Disabled | Enabled
      mask TypeOptions ADC_FIFO_6: 0 | 1 | 2 | 3 | 4 | 5 | 6 | 7
      mask TypeOptions ADC_CHA_6: 0 | 1 | 2 | 3 | 4 | 5 | 6 | 7 | 8 | 9 | 10 | 11 | 12 | 13 | 14 | 15
      mask TypeOptions ADC_CHB_6: 0 | 1 | 2 | 3 | 4 | 5 | 6 | 7 | 8 | 9 | 10 | 11 | 12 | 13 | 14 | 15
      mask TypeOptions ADC_CMS_7: Single-conversion mode: ADC unit A | Single-conversion mode: ADC unit B | Dual-conversion mode
      mask TypeOptions ADC_CIR_7: Disabled | Enabled
      mask TypeOptions ADC_FIFO_7: 0 | 1 | 2 | 3 | 4 | 5 | 6 | 7
      mask TypeOptions ADC_CHA_7: 0 | 1 | 2 | 3 | 4 | 5 | 6 | 7 | 8 | 9 | 10 | 11 | 12 | 13 | 14 | 15
      mask TypeOptions ADC_CHB_7: 0 | 1 | 2 | 3 | 4 | 5 | 6 | 7 | 8 | 9 | 10 | 11 | 12 | 13 | 14 | 15
      mask TypeOptions ADC_CMS_8: Single-conversion mode: ADC unit A | Single-conversion mode: ADC unit B | Dual-conversion mode
      mask TypeOptions ADC_CIR_8: Disabled | Enabled
      mask TypeOptions ADC_FIFO_8: 0 | 1 | 2 | 3 | 4 | 5 | 6 | 7
      mask TypeOptions ADC_CHA_8: 0 | 1 | 2 | 3 | 4 | 5 | 6 | 7 | 8 | 9 | 10 | 11 | 12 | 13 | 14 | 15
      mask TypeOptions ADC_CHB_8: 0 | 1 | 2 | 3 | 4 | 5 | 6 | 7 | 8 | 9 | 10 | 11 | 12 | 13 | 14 | 15
      mask TypeOptions ADC_CMS_9: Single-conversion mode: ADC unit A | Single-conversion mode: ADC unit B | Dual-conversion mode
      mask TypeOptions ADC_CIR_9: Disabled | Enabled
      mask TypeOptions ADC_FIFO_9: 0 | 1 | 2 | 3 | 4 | 5 | 6 | 7
      mask TypeOptions ADC_CHA_9: 0 | 1 | 2 | 3 | 4 | 5 | 6 | 7 | 8 | 9 | 10 | 11 | 12 | 13 | 14 | 15
      mask TypeOptions ADC_CHB_9: 0 | 1 | 2 | 3 | 4 | 5 | 6 | 7 | 8 | 9 | 10 | 11 | 12 | 13 | 14 | 15
      mask TypeOptions ADC_CMS_10: Single-conversion mode: ADC unit A | Single-conversion mode: ADC unit B | Dual-conversion mode
      mask TypeOptions ADC_CIR_10: Disabled | Enabled
      mask TypeOptions ADC_FIFO_10: 0 | 1 | 2 | 3 | 4 | 5 | 6 | 7
      mask TypeOptions ADC_CHA_10: 0 | 1 | 2 | 3 | 4 | 5 | 6 | 7 | 8 | 9 | 10 | 11 | 12 | 13 | 14 | 15
      mask TypeOptions ADC_CHB_10: 0 | 1 | 2 | 3 | 4 | 5 | 6 | 7 | 8 | 9 | 10 | 11 | 12 | 13 | 14 | 15
      mask TypeOptions ADC_CMS_11: Single-conversion mode: ADC unit A | Single-conversion mode: ADC unit B | Dual-conversion mode
      mask TypeOptions ADC_CIR_11: Disabled | Enabled
      mask TypeOptions ADC_FIFO_11: 0 | 1 | 2 | 3 | 4 | 5 | 6 | 7
      mask TypeOptions ADC_CHA_11: 0 | 1 | 2 | 3 | 4 | 5 | 6 | 7 | 8 | 9 | 10 | 11 | 12 | 13 | 14 | 15
      mask TypeOptions ADC_CHB_11: 0 | 1 | 2 | 3 | 4 | 5 | 6 | 7 | 8 | 9 | 10 | 11 | 12 | 13 | 14 | 15
      mask TypeOptions ADC_CMS_12: Single-conversion mode: ADC unit A | Single-conversion mode: ADC unit B | Dual-conversion mode
      mask TypeOptions ADC_CIR_12: Disabled | Enabled
      mask TypeOptions ADC_FIFO_12: 0 | 1 | 2 | 3 | 4 | 5 | 6 | 7
      mask TypeOptions ADC_CHA_12: 0 | 1 | 2 | 3 | 4 | 5 | 6 | 7 | 8 | 9 | 10 | 11 | 12 | 13 | 14 | 15
      mask TypeOptions ADC_CHB_12: 0 | 1 | 2 | 3 | 4 | 5 | 6 | 7 | 8 | 9 | 10 | 11 | 12 | 13 | 14 | 15
      mask TypeOptions ADC_CMS_13: Single-conversion mode: ADC unit A | Single-conversion mode: ADC unit B | Dual-conversion mode
      mask TypeOptions ADC_CIR_13: Disabled | Enabled
      mask TypeOptions ADC_FIFO_13: 0 | 1 | 2 | 3 | 4 | 5 | 6 | 7
      mask TypeOptions ADC_CHA_13: 0 | 1 | 2 | 3 | 4 | 5 | 6 | 7 | 8 | 9 | 10 | 11 | 12 | 13 | 14 | 15
      mask TypeOptions ADC_CHB_13: 0 | 1 | 2 | 3 | 4 | 5 | 6 | 7 | 8 | 9 | 10 | 11 | 12 | 13 | 14 | 15
      mask TypeOptions ADC_CMS_14: Single-conversion mode: ADC unit A | Single-conversion mode: ADC unit B | Dual-conversion mode
      mask TypeOptions ADC_CIR_14: Disabled | Enabled
      mask TypeOptions ADC_FIFO_14: 0 | 1 | 2 | 3 | 4 | 5 | 6 | 7
      mask TypeOptions ADC_CHA_14: 0 | 1 | 2 | 3 | 4 | 5 | 6 | 7 | 8 | 9 | 10 | 11 | 12 | 13 | 14 | 15
      mask TypeOptions ADC_CHB_14: 0 | 1 | 2 | 3 | 4 | 5 | 6 | 7 | 8 | 9 | 10 | 11 | 12 | 13 | 14 | 15
      mask TypeOptions ADC_CMS_15: Single-conversion mode: ADC unit A | Single-conversion mode: ADC unit B | Dual-conversion mode
      mask TypeOptions ADC_CIR_15: Disabled | Enabled
      mask TypeOptions ADC_FIFO_15: 0 | 1 | 2 | 3 | 4 | 5 | 6 | 7
      mask TypeOptions ADC_CHA_15: 0 | 1 | 2 | 3 | 4 | 5 | 6 | 7 | 8 | 9 | 10 | 11 | 12 | 13 | 14 | 15
      mask TypeOptions ADC_CHB_15: 0 | 1 | 2 | 3 | 4 | 5 | 6 | 7 | 8 | 9 | 10 | 11 | 12 | 13 | 14 | 15
      mask TypeOptions ADC_CMS_16: Single-conversion mode: ADC unit A | Single-conversion mode: ADC unit B | Dual-conversion mode
      mask TypeOptions ADC_CIR_16: Disabled | Enabled
      mask TypeOptions ADC_FIFO_16: 0 | 1 | 2 | 3 | 4 | 5 | 6 | 7
      mask TypeOptions ADC_CHA_16: 0 | 1 | 2 | 3 | 4 | 5 | 6 | 7 | 8 | 9 | 10 | 11 | 12 | 13 | 14 | 15
      mask TypeOptions ADC_CHB_16: 0 | 1 | 2 | 3 | 4 | 5 | 6 | 7 | 8 | 9 | 10 | 11 | 12 | 13 | 14 | 15
      mask TypeOptions ADC_CMS_17: Single-conversion mode: ADC unit A | Single-conversion mode: ADC unit B | Dual-conversion mode
      mask TypeOptions ADC_CIR_17: Disabled | Enabled
      mask TypeOptions ADC_FIFO_17: 0 | 1 | 2 | 3 | 4 | 5 | 6 | 7
      mask TypeOptions ADC_CHA_17: 0 | 1 | 2 | 3 | 4 | 5 | 6 | 7 | 8 | 9 | 10 | 11 | 12 | 13 | 14 | 15
      mask TypeOptions ADC_CHB_17: 0 | 1 | 2 | 3 | 4 | 5 | 6 | 7 | 8 | 9 | 10 | 11 | 12 | 13 | 14 | 15
      mask TypeOptions ADC_CMS_18: Single-conversion mode: ADC unit A | Single-conversion mode: ADC unit B | Dual-conversion mode
      mask TypeOptions ADC_CIR_18: Disabled | Enabled
      mask TypeOptions ADC_FIFO_18: 0 | 1 | 2 | 3 | 4 | 5 | 6 | 7
      mask TypeOptions ADC_CHA_18: 0 | 1 | 2 | 3 | 4 | 5 | 6 | 7 | 8 | 9 | 10 | 11 | 12 | 13 | 14 | 15
      mask TypeOptions ADC_CHB_18: 0 | 1 | 2 | 3 | 4 | 5 | 6 | 7 | 8 | 9 | 10 | 11 | 12 | 13 | 14 | 15
      mask TypeOptions ADC_CMS_19: Single-conversion mode: ADC unit A | Single-conversion mode: ADC unit B | Dual-conversion mode
      mask TypeOptions ADC_CIR_19: Disabled | Enabled
      mask TypeOptions ADC_FIFO_19: 0 | 1 | 2 | 3 | 4 | 5 | 6 | 7
      mask TypeOptions ADC_CHA_19: 0 | 1 | 2 | 3 | 4 | 5 | 6 | 7 | 8 | 9 | 10 | 11 | 12 | 13 | 14 | 15
      mask TypeOptions ADC_CHB_19: 0 | 1 | 2 | 3 | 4 | 5 | 6 | 7 | 8 | 9 | 10 | 11 | 12 | 13 | 14 | 15
      mask TypeOptions ADC_CMS_20: Single-conversion mode: ADC unit A | Single-conversion mode: ADC unit B | Dual-conversion mode
      mask TypeOptions ADC_CIR_20: Disabled | Enabled
      mask TypeOptions ADC_FIFO_20: 0 | 1 | 2 | 3 | 4 | 5 | 6 | 7
      mask TypeOptions ADC_CHA_20: 0 | 1 | 2 | 3 | 4 | 5 | 6 | 7 | 8 | 9 | 10 | 11 | 12 | 13 | 14 | 15
      mask TypeOptions ADC_CHB_20: 0 | 1 | 2 | 3 | 4 | 5 | 6 | 7 | 8 | 9 | 10 | 11 | 12 | 13 | 14 | 15
      mask TypeOptions ADC_CMS_21: Single-conversion mode: ADC unit A | Single-conversion mode: ADC unit B | Dual-conversion mode
      mask TypeOptions ADC_CIR_21: Disabled | Enabled
      mask TypeOptions ADC_FIFO_21: 0 | 1 | 2 | 3 | 4 | 5 | 6 | 7
      mask TypeOptions ADC_CHA_21: 0 | 1 | 2 | 3 | 4 | 5 | 6 | 7 | 8 | 9 | 10 | 11 | 12 | 13 | 14 | 15
      mask TypeOptions ADC_CHB_21: 0 | 1 | 2 | 3 | 4 | 5 | 6 | 7 | 8 | 9 | 10 | 11 | 12 | 13 | 14 | 15
      mask TypeOptions ADC_CMS_22: Single-conversion mode: ADC unit A | Single-conversion mode: ADC unit B | Dual-conversion mode
      mask TypeOptions ADC_CIR_22: Disabled | Enabled
      mask TypeOptions ADC_FIFO_22: 0 | 1 | 2 | 3 | 4 | 5 | 6 | 7
      mask TypeOptions ADC_CHA_22: 0 | 1 | 2 | 3 | 4 | 5 | 6 | 7 | 8 | 9 | 10 | 11 | 12 | 13 | 14 | 15
      mask TypeOptions ADC_CHB_22: 0 | 1 | 2 | 3 | 4 | 5 | 6 | 7 | 8 | 9 | 10 | 11 | 12 | 13 | 14 | 15
      mask TypeOptions ADC_CMS_23: Single-conversion mode: ADC unit A | Single-conversion mode: ADC unit B | Dual-conversion mode
      mask TypeOptions ADC_CIR_23: Disabled | Enabled
      mask TypeOptions ADC_FIFO_23: 0 | 1 | 2 | 3 | 4 | 5 | 6 | 7
      mask TypeOptions ADC_CHA_23: 0 | 1 | 2 | 3 | 4 | 5 | 6 | 7 | 8 | 9 | 10 | 11 | 12 | 13 | 14 | 15
      mask TypeOptions ADC_CHB_23: 0 | 1 | 2 | 3 | 4 | 5 | 6 | 7 | 8 | 9 | 10 | 11 | 12 | 13 | 14 | 15
      mask TypeOptions ADC_CMS_24: Single-conversion mode: ADC unit A | Single-conversion mode: ADC unit B | Dual-conversion mode
      mask TypeOptions ADC_CIR_24: Disabled | Enabled
      mask TypeOptions ADC_FIFO_24: 0 | 1 | 2 | 3 | 4 | 5 | 6 | 7
      mask TypeOptions ADC_CHA_24: 0 | 1 | 2 | 3 | 4 | 5 | 6 | 7 | 8 | 9 | 10 | 11 | 12 | 13 | 14 | 15
      mask TypeOptions ADC_CHB_24: 0 | 1 | 2 | 3 | 4 | 5 | 6 | 7 | 8 | 9 | 10 | 11 | 12 | 13 | 14 | 15
      mask Callback dst:
      | CTU_unit.init();
      | disp_string = CTU_unit.display_st;
      | set_param(gcb,'dst',disp_string);
      mask TypeOptions T0_ADC_CMS_1: Single-conversion mode: ADC unit A | Single-conversion mode: ADC unit B | Dual-conversion mode
      mask TypeOptions T0_ADC_CIR_1: Disabled | Enabled
      mask TypeOptions T0_ADC_FIFO_1: 0 | 1 | 2 | 3 | 4 | 5 | 6 | 7
      mask TypeOptions T0_ADC_CHA_1: 0 | 1 | 2 | 3 | 4 | 5 | 6 | 7 | 8 | 9 | 10 | 11 | 12 | 13 | 14 | 15
      mask TypeOptions T0_ADC_CHB_1: 0 | 1 | 2 | 3 | 4 | 5 | 6 | 7 | 8 | 9 | 10 | 11 | 12 | 13 | 14 | 15
      mask TypeOptions T0_ADC_CMS_2: Single-conversion mode: ADC unit A | Single-conversion mode: ADC unit B | Dual-conversion mode
      mask TypeOptions T0_ADC_CIR_2: Disabled | Enabled
      mask TypeOptions T0_ADC_FIFO_2: 0 | 1 | 2 | 3 | 4 | 5 | 6 | 7
      mask TypeOptions T0_ADC_CHA_2: 0 | 1 | 2 | 3 | 4 | 5 | 6 | 7 | 8 | 9 | 10 | 11 | 12 | 13 | 14 | 15
      mask TypeOptions T0_ADC_CHB_2: 0 | 1 | 2 | 3 | 4 | 5 | 6 | 7 | 8 | 9 | 10 | 11 | 12 | 13 | 14 | 15
      mask TypeOptions T0_ADC_CMS_3: Single-conversion mode: ADC unit A | Single-conversion mode: ADC unit B | Dual-conversion mode
      mask TypeOptions T0_ADC_CIR_3: Disabled | Enabled
      mask TypeOptions T0_ADC_FIFO_3: 0 | 1 | 2 | 3 | 4 | 5 | 6 | 7
      mask TypeOptions T0_ADC_CHA_3: 0 | 1 | 2 | 3 | 4 | 5 | 6 | 7 | 8 | 9 | 10 | 11 | 12 | 13 | 14 | 15
      mask TypeOptions T0_ADC_CHB_3: 0 | 1 | 2 | 3 | 4 | 5 | 6 | 7 | 8 | 9 | 10 | 11 | 12 | 13 | 14 | 15
      mask TypeOptions T1_ADC_CMS_1: Single-conversion mode: ADC unit A | Single-conversion mode: ADC unit B | Dual-conversion mode
      mask TypeOptions T1_ADC_CIR_1: Disabled | Enabled
      mask TypeOptions T1_ADC_FIFO_1: 0 | 1 | 2 | 3 | 4 | 5 | 6 | 7
      mask TypeOptions T1_ADC_CHA_1: 0 | 1 | 2 | 3 | 4 | 5 | 6 | 7 | 8 | 9 | 10 | 11 | 12 | 13 | 14 | 15
      mask TypeOptions T1_ADC_CHB_1: 0 | 1 | 2 | 3 | 4 | 5 | 6 | 7 | 8 | 9 | 10 | 11 | 12 | 13 | 14 | 15
      mask TypeOptions T1_ADC_CMS_2: Single-conversion mode: ADC unit A | Single-conversion mode: ADC unit B | Dual-conversion mode
      mask TypeOptions T1_ADC_CIR_2: Disabled | Enabled
      mask TypeOptions T1_ADC_FIFO_2: 0 | 1 | 2 | 3 | 4 | 5 | 6 | 7
      mask TypeOptions T1_ADC_CHA_2: 0 | 1 | 2 | 3 | 4 | 5 | 6 | 7 | 8 | 9 | 10 | 11 | 12 | 13 | 14 | 15
      mask TypeOptions T1_ADC_CHB_2: 0 | 1 | 2 | 3 | 4 | 5 | 6 | 7 | 8 | 9 | 10 | 11 | 12 | 13 | 14 | 15
      mask TypeOptions T1_ADC_CMS_3: Single-conversion mode: ADC unit A | Single-conversion mode: ADC unit B | Dual-conversion mode
      mask TypeOptions T1_ADC_CIR_3: Disabled | Enabled
      mask TypeOptions T1_ADC_FIFO_3: 0 | 1 | 2 | 3 | 4 | 5 | 6 | 7
      mask TypeOptions T1_ADC_CHA_3: 0 | 1 | 2 | 3 | 4 | 5 | 6 | 7 | 8 | 9 | 10 | 11 | 12 | 13 | 14 | 15
      mask TypeOptions T1_ADC_CHB_3: 0 | 1 | 2 | 3 | 4 | 5 | 6 | 7 | 8 | 9 | 10 | 11 | 12 | 13 | 14 | 15
      mask Display: disp(st);
  CTU ISR : S-Function  Priority=2  FunctionName=CTU_564xl_interrupt  Parameters=outMask,uint16(intSrc)  SFunctionDeploymentMode=off  EnableBusSupport=off  mask(CTU_564xL_interrupt){intSource=Trigger interrupt, intSrc=128, Trigger=0, isrPriority=12, isrPrio=12, outMask=off}
      mask prompts: intSource "Interrupt source"; isrPriority "Priority"; isrPrio "priority"; outMask "Mask"
      mask help: CTU interrupt
      mask init:
      | isrPr = get_param(gcb,'isrPriority');
      | src = get_param (gcb,'intSource');
      | trig = get_param (gcb,'Trigger'); 
      | 
      | set_param(gcb,'isrPrio',num2str(isrPr));
      | 
      | crlf= sprintf('\n');
      | ctuir = 0;
      | srcStr = src;
      | set_param(gcb,'outMask','off');
      | 
      | if strcmp (src, 'Trigger interrupt')
      |    srcStr = ['Trigger ', trig,' interrupt'];
      |    ctuir = bitset(uint16(ctuir),7-str2num(trig)+1);
      | elseif strcmp (src, 'MRS interrupt')
      |    ctuir = bitset(uint16(ctuir),14+1);
      | elseif strcmp (src, 'Error interrupt')
      |    ctuir = bitset(uint16(ctuir),15+1);
      |    set_param(gcb,'outMask','on');
      | end
      | set_param(gcb,'intSrc',num2str(ctuir));
      | 
      | st=[srcStr,crlf,'ISR priority: ',isrPr];
      mask Help: web([rappid_block_help,filesep,'CTU_ISR.htm']);
      mask TypeOptions intSource: Trigger interrupt | MRS interrupt | Error interrupt | ADC command interrupt
      mask Callback intSource:
      | MaskVisibilities = get_param(gcb,'MaskVisibilities');
      | if strcmp (get_param (gcb, 'intSource'), 'Trigger interrupt')
      |    MaskVisibilities{3} = 'on';
      | else
      |    MaskVisibilities{3} = 'off';
      | end
      | set_param(gcb,'MaskVisibilities',MaskVisibilities);
      mask TypeOptions Trigger: 0 | 1 | 2 | 3 | 4 | 5 | 6 | 7
      mask TypeOptions isrPriority: 0 | 1 | 2 | 3 | 4 | 5 | 6 | 7 | 8 | 9 | 10 | 11 | 12 | 13 | 14 | 15
      mask Display:
      | disp(st);
      | port_label('output',1, 'trigger')
  CTU ISR enable-disable : S-Function  Priority=2  FunctionName=CTU_564xl_disable_interrupt  Parameters=uint16(intSrc)  SFunctionDeploymentMode=off  EnableBusSupport=off  mask(CTU_564xL_disable_interrupt){intSrc=0, Trigger0=off, Trigger1=off, Trigger2=off, Trigger3=off, Trigger4=off, Trigger5=off, Trigger6=off, Trigger7=off, msr=off, error=off}
      mask prompts: Trigger0 "Enable Trigger 0 interrupt"; Trigger1 "Enable Trigger 1 interrupt"; Trigger2 "Enable Trigger 2 interrupt"; Trigger3 "Enable Trigger 3 interrupt"; Trigger4 "Enable Trigger 4 interrupt"; Trigger5 "Enable Trigger 5 interrupt"; Trigger6 "Enable Trigger 6 interrupt"; Trigger7 "Enable Trigger 7 interrupt"; msr "Enable MRS interrupt"; error "Enable Error interrupt"
      mask help: CTU interrupt enable/disable
      mask init:
      | crlf= sprintf('\n');
      | ctuir = 0;
      | 
      | for i = 0:7
      |     if (strcmp(get_param (gcb, ['Trigger',num2str(i)]),'on'))
      |         ctuir = bitset(uint16(ctuir),8+i+1);
      |     end
      | end
      | if (strcmp(get_param (gcb, 'msr'),'on'))
      |     ctuir = bitset(uint16(ctuir),2);
      | end
      | if (strcmp(get_param (gcb, 'error'),'on'))
      |     ctuir = bitset(uint16(ctuir),1);
      | end
      | set_param(gcb,'intSrc',num2str(ctuir));
      | 
      | st=['Interrupt Enable (CTUIR): ',dec2bin(ctuir,16)];
      mask Help: web([rappid_block_help,filesep,'CTU_ISR_enable.htm']);
      mask Display: disp(st);
  Complementary PWM Output : S-Function  Priority=1  FunctionName=Comp_PWM_564xL_output  Parameters=pwmMod,subMod,uint32(InitFreq),uint16(InitDuty),uint16(DeadTime),pcrNumA,pcrNumB,pwm45en,uint16(InitDutyB),uint16(outTrig),masterSync,debug_mode,deadtime_mks,uint16(octrl),resValue  SFunctionDeploymentMode=off  EnableBusSupport=off  mask(Comp_PWM_564xL_output){pwmModule=0, pwmMod=0, SubModule=0, subMod=0, InitFreq=0, resolution=1 %, resValue=1, InitDuty=0, pwm45=off, pwm45en=0, InitDutyB=0, DeadTime=0, dt=IPBus clock cycles, deadtime_mks=0, debugSw=on, debug_mode=1, pin_A0=None, pin_B0=None, pin_A1=None, pin_B1=None, pin_A2=None, pin_B2=None, pin_A3=None, pin_B3=None, pin1_A0=None, pin1_B0=None, pin1_A1=None, pin1_B1=None, pin1_A2=None, pin1_B2=None, pin1_A3=None, pin1_B3=None, pcrNumA=255, pcrNumB=255, polA=off, polB=off, octrl=0, syncFrom0=off, masterSync=0, outVal0=off, outVal1=off, outVal2=on, outVal3=on, outVal4=on, outVal5=on, outTrig=12}
      mask prompts: pwmModule "Module"; pwmMod "Module"; SubModule "Submodule (0-3)"; subMod "subModule (0 - 3)"; InitFreq "Initial Frequency, Hz"; resValue "Resolution"; InitDuty "PWM23: initial DutyCycle A and B (0..100)"; pwm45 "PWM45 for Output Trigger"; pwm45en "PWM45 for Output Trigger"; InitDutyB "PWM45: initial DutyCycle (0..100)"; DeadTime "Initial Deadtime"; dt "Deadtime values in"; debugSw "Duty Cycle Simulation output"; debug_mode "Duty Cycle Simulation output"; pin_A0 "A[0] output pin"; pin_B0 "B[0] output pin"; pin_A1 "A[1] output pin"; pin_B1 "B[1] output pin"; pin_A2 "A[2] output pin"; pin_B2 "B[2] output pin"; pin_A3 "A[3] output pin"; pin_B3 "B[3] output pin"; pin1_A0 "A[0] output pin"; pin1_B0 "B[0] output pin"; pin1_A1 "A[1] output pin"; pin1_B1 "B[1] output pin"; pin1_A2 "A[2] output pin"; pin1_B2 "B[2] output pin"; pin1_A3 "A[3] output pin"; pin1_B3 "B[3] output pin"; polA "Invert PWMA Output Polarity"; polB "Invert PWMB Output Polarity"; syncFrom0 "Counter synchronization from Submodule 0"; masterSync "Counter synchronization"; outVal0 "VAL0"; outVal1 "VAL1"; outVal2 "VAL2"; outVal3 "VAL3"; outVal4 "VAL4"; outVal5 "VAL5"; outTrig "Output Trigger"
      mask help: Two Channel Complementary PWM output with deadtime insertion per channel with frequency and duty cycle input control.
      mask init:
      | PwmMod = get_param(gcb,'pwmModule');
      | SubMod = get_param(gcb,'SubModule');
      | 
      | crlf= sprintf('\n');
      | st = [''];
      | labels = [];
      | str_disp = 'disp(st);';
      | 
      | str_pi1 = 'port_label(''input'',1,''Frequency'')';
      | str_pi2 = 'port_label(''input'',2,''Duty Cycle A,B'')';
      | str_pi3 = 'port_label(''input'',3,''PWM A Deadtime'')';
      | str_pi4 = 'port_label(''input'',4,''PWM B Deadtime'')';
      | str_pi5 = 'port_label(''input'',5,''Duty Cycle PWM45'')';
      | 
      | str_po1 = 'port_label(''output'',1,''Duty Cycle A,B'')';
      | 
      | r = get_param(gcb,'resolution');
      | if isempty(strfind(r,'.001'))==0
      |   res = 1000;
      | elseif isempty(strfind(r,'.01'))==0
      |   res = 100;
      | elseif isempty(strfind(r,'.1'))==0
      |   res = 10;
      | else
      |   res = 1;
      | end
      | set_param(gcb,'resValue',num2str(res));
      | 
      | freq = num2str(get_param(gcb,'InitFreq'));
      | duty = num2str(str2num(get_param(gcb,'InitDuty'))/res);
      | dt = num2str(get_param(gcb,'DeadTime'));
      | mod = num2str(SubMod);
      | set_param(gcb,'subMod',mod);
      | 
      | pwm_m = num2str(PwmMod);
      | set_param(gcb,'pwmMod',pwm_m);
      | if strcmp(pwm_m,'0')==0
      |     pwmStr = pwm_m;
      | else
      |     pwmStr = '';
      | end
      | 
      | pcrStr = get_param(gcb,['pin',pwmStr,'_A',mod]);
      | if strcmp(pcrStr,'None')==1
      |    set_param(gcb,'pcrNumA','255');
      | else    
      |    posColon = findstr(pcrStr, ':');
      |    num = strtrim(pcrStr(1:posColon(1)-1));
      |    set_param(gcb,'pcrNumA',num);
      | end
      | 
      | pcrStr = get_param(gcb,['pin',pwmStr,'_B',mod]);
      | if strcmp(pcrStr,'None')==1
      |    set_param(gcb,'pcrNumB','255');
      | else    
      |    posColon = findstr(pcrStr, ':');
      |    num = strtrim(pcrStr(1:posColon(1)-1));
      |    set_param(gcb,'pcrNumB',num);
      | end
      | 
      | if strcmp(get_param(gcb,'debugSw'),'on')==1,
      |    debug_mode = 1;   
      |    set_param(gcb,'debug_mode','1');
      |    labels = [labels str_po1 char(10)];
      | else
      |    debug_mode = 0;   
      |    set_param(gcb,'debug_mode','0');
      | end
      | 
      | if strcmp(get_param(gcb,'pwm45'),'on')==1,
      |    pwm45en = 1;
      |    set_param(gcb,'pwm45en','1');
      |    labels = [labels str_pi5 char(10)];
      |    maxTrig = 5;
      | else
      |    pwm45en = 0;
      |    set_param(gcb,'pwm45en','0');
      |    maxTrig = 3;
      | end
      | 
      | if strcmp(get_param(gcb,'dt'),'microseconds')==1,
      |    set_param(gcb,'deadtime_mks','1');
      |    dt_str = ' microseconds';
      | else
      |    set_param(gcb,'deadtime_mks','0');
      |    dt_str = ' IPBus cycles';
      | end
      | 
      | st=['PWM Module: ',PwmMod,'   Sub Module ',SubMod ,crlf,...
      |     ' Initial Frequency  ',freq,'Hz',crlf,...
      |     ' Initial DutyCycle ',duty,'% ',crlf,' Initial DeadTime ',dt,dt_str];
      | 
      | labels = [labels str_disp char(10)];
      | labels = [labels str_pi1 char(10)];
      | labels = [labels str_pi2 char(10)];
      | labels = [labels str_pi3 char(10)];
      | labels = [labels str_pi4 char(10)];
      | 
      | labels(end) = [];
      | set_param(gcb,'MaskDisplay',labels);
      | 
      | outT = 0;
      | for i = 0:maxTrig
      |     if (strcmp(get_param (gcb, ['outVal',num2str(i)]),'on'))
      |          outT = bitset(uint16(outT),i+1);
      |     end
      | end
      | set_param(gcb,'outTrig',num2str(outT));
      | 
      | if strcmp(get_param(gcb,'syncFrom0'),'on')==1,
      |    set_param(gcb,'masterSync','1');
      | else
      |    set_param(gcb,'masterSync','0');
      | end
      | 
      | polarityAB = 0;
      | if strcmp(get_param(gcb,'polA'),'on')==1,
      |    polarityAB = bitset(uint16(polarityAB),11);
      | end
      | if strcmp(get_param(gcb,'polB'),'on')==1,
      |    polarityAB = bitset(uint16(polarityAB),10);
      | end
      | set_param(gcb,'octrl',num2str(polarityAB));
      mask Help: web([rappid_block_help,filesep,'Comp_PWM_output.htm']);
      mask TypeOptions pwmModule: 0 | 1
      mask Callback pwmModule: rappid_564xl_block_pwm_change_mod (gcb,17,2,38);
      mask TypeOptions SubModule: 0 | 1 | 2 | 3
      mask Callback SubModule: rappid_564xl_block_pwm_change_mod (gcb,17,2,38);
      mask TypeOptions resolution: 1 % | 0.1 % | 0.01 % | 0.001 %
      mask Callback resolution:
      | MaskPrompts = get_param(gcb,'MaskPrompts');
      | r = get_param(gcb,'resolution');
      | if isempty(strfind(r,'.001'))==0
      |   mStr = regexprep(MaskPrompts{8},'..\d+\)','..100000)');
      |   if strcmp(mStr,MaskPrompts{8})==0
      |      MaskPrompts{8} = regexprep(MaskPrompts{8},'..\d+\)','..100000)');
      |      MaskPrompts{11} = regexprep(MaskPrompts{11},'..\d+\)','..100000)');
      |      set_param(gcb,'MaskPrompts',MaskPrompts);
      |   end
      | elseif isempty(strfind(r,'.01'))==0
      |   mStr = regexprep(MaskPrompts{8},'..\d+\)','..10000)');
      |   if strcmp(mStr,MaskPrompts{8})==0
      |      MaskPrompts{8} = regexprep(MaskPrompts{8},'..\d+\)','..10000)');
      |      MaskPrompts{11} = regexprep(MaskPrompts{11},'..\d+\)','..10000)');
      |      set_param(gcb,'MaskPrompts',MaskPrompts);
      |   end
      | elseif isempty(strfind(r,'.1'))==0
      |   mStr = regexprep(MaskPrompts{8},'..\d+\)','..1000)');
      |   if strcmp(mStr,MaskPrompts{8})==0
      |      MaskPrompts{8} = regexprep(MaskPrompts{8},'..\d+\)','..1000)');
      |      MaskPrompts{11} = regexprep(MaskPrompts{11},'..\d+\)','..1000)');
      |      set_param(gcb,'MaskPrompts',MaskPrompts);
      |   end
      | else
      |   mStr = regexprep(MaskPrompts{8},'..\d+\)','..100)');
      |   if strcmp(mStr,MaskPrompts{8})==0
      |      MaskPrompts{8} = regexprep(MaskPrompts{8},'..\d+\)','..100)');
      |      MaskPrompts{11} = regexprep(MaskPrompts{11},'..\d+\)','..100)');
      |      set_param(gcb,'MaskPrompts',MaskPrompts);
      |   end
      | end
      mask Callback pwm45:
      | MaskVisibilities = get_param(gcb,'MaskVisibilities');
      | if strcmp(get_param(gcb,'pwm45'),'on')==1,
      |     MaskVisibilities{11} = 'on';
      |     MaskVisibilities{44} = 'on';
      |     MaskVisibilities{45} = 'on';
      | else
      |     MaskVisibilities{11} = 'off';
      |     MaskVisibilities{44} = 'off';
      |     MaskVisibilities{45} = 'off';
      | end
      | set_param(gcb,'MaskVisibilities',MaskVisibilities);
      mask TypeOptions dt: IPBus clock cycles | microseconds
      mask TypeOptions pin_A0: None | 11  : PA11 : [ 120 ] : [ D11 ] | 58  : PD10 : [ 76 ] : [ T15 ]
      mask TypeOptions pin_B0: None | 10  : PA10 : [ 118 ] : [A13 ] | 59  : PD11 : [ 78 ] : [ R16 ]
      mask TypeOptions pin_A1: None | 39  : PC7  : [ 15 ] : [ K4 ] | 47  : PC15 : [ 124 ] : [ A8 ] | 80  : PF0  : [ 133 ] : [ D7 ]
      mask TypeOptions pin_B1: None | 38  : PC6  : [ 142 ] : [ D4 ] | 48  : PD0  : [ 125 ] : [ B8 ] | 62  : PD14 : [ 105 ] : [ D16 ]
      mask TypeOptions pin_A2: None | 11  : PA11 : [ 120 ] : [ D11 ] | 12  : PA12 : [ 122 ] : [ A10 ] | 99  : PG3  : [ 104 ] : [ D17 ]
      mask TypeOptions pin_B2: None | 12  : PA12 : [ 122 ] : [ A10 ] | 13  : PA13 : [ 136 ] : [ C6 ] | 100 : PG4  : [ 100 ] : [ F17 ]
      mask TypeOptions pin_A3: None | 2   : PA2  : [ 84 ] : [ N16 ] | 42  : PC10 : [ 111 ] : [ A15 ] | 51  : PD3  : [ 128 ] : [ A7 ] | 102 : PG6  : [ 98 ] : [ G17 ]
      mask TypeOptions pin_B3: None | 3   : PA3  : [ 92 ] : [ K17 ] | 9   : PA9  : [ 134 ] : [ B6 ] | 52  : PD4  : [ 129 ] : [ B7 ] | 103 : PG7  : [ 83 ] : [ P17 ]
      mask TypeOptions pin1_A0: None | 117 : PH5 : [ --- ] : [ M17 ]
      mask TypeOptions pin1_B0: None | 118 : PH6 : [ --- ] : [ H17 ]
      mask TypeOptions pin1_A1: None | 120 : PH8 : [ --- ] : [ K15 ]
      mask TypeOptions pin1_B1: None | 121 : PH9 : [ --- ] : [ G16 ]
      mask TypeOptions pin1_A2: None | 123 : PH11 : [ --- ] : [ C11 ]
      mask TypeOptions pin1_B2: None | 124 : PH12 : [ --- ] : [ B10 ]
      mask TypeOptions pin1_A3: None | 126 : PH14 : [ --- ] : [ A12 ]
      mask TypeOptions pin1_B3: None | 127 : PH15 : [ --- ] : [ J17 ]
      mask Display:
      | port_label('output',1,'Duty Cycle A,B')
      | disp(st);
      | port_label('input',1,'Frequency')
      | port_label('input',2,'Duty Cycle A,B')
      | port_label('input',3,'PWM A Deadtime')
      | port_label('input',4,'PWM B Deadtime')
  FlexPWM ISR : S-Function  Priority=2  FunctionName=pwm_564xl_interrupt  Parameters=outMask,uint16(intSrc),uint16(subMod),uint16(isrPrio),uint16(pwmMod)  SFunctionDeploymentMode=off  EnableBusSupport=off  mask(PWM_564xL_interrupt){intSource=Compare interrupt, intSrc=63, Module=0, pwmMod=0, SubModule=0, subMod=0, val0=on, val1=on, val2=on, val3=on, val4=on, val5=on, isrPriority=12, isrPrio=12, outMask=on}
      mask prompts: intSource "Interrupt source"; intSrc "int source"; pwmMod "mod"; isrPriority "Priority"; isrPrio "priority"; outMask "Mask"
      mask help: FlexPWM interrupt
      mask init:
      | Mod = get_param(gcb,'Module');
      | SubMod = get_param(gcb,'SubModule');
      | isrPr = get_param(gcb,'isrPriority');
      | src = get_param (gcb,'intSource');
      | 
      | set_param(gcb,'pwmMod',num2str(Mod));
      | set_param(gcb,'subMod',num2str(SubMod));
      | set_param(gcb,'isrPrio',num2str(isrPr));
      | 
      | crlf= sprintf('\n');
      | srcStr = ['PWM Module: ',Mod,'   Sub Module: ',SubMod,crlf];
      | cmpf = 0;
      | set_param(gcb,'outMask','off');
      | 
      | if strcmp (src, 'Compare interrupt')
      |    for i = 0:5
      |        if (strcmp(get_param (gcb, ['val',num2str(i)]),'on'))
      |             cmpf = bitset(uint16(cmpf),i+1);
      |        end
      |    end
      |    set_param(gcb,'outMask','on');
      | elseif strcmp (src, 'Reload interrupt')
      |    cmpf = bitset(uint16(cmpf),12+1);
      | elseif strcmp (src, 'Reload error interrupt')
      |    cmpf = bitset(uint16(cmpf),13+1);
      | end
      | set_param(gcb,'intSrc',num2str(cmpf));
      | 
      | st=[src,crlf,srcStr,'ISR priority: ',isrPr];
      mask Help: web([rappid_block_help,filesep,'PWM_ISR.htm']);
      mask TypeOptions intSource: Compare interrupt | Reload interrupt | Reload error interrupt
      mask Callback intSource:
      | MaskVisibilities = get_param(gcb,'MaskVisibilities');
      | if strcmp (get_param (gcb, 'intSource'), 'Compare interrupt')
      |    for i=7:12
      |         MaskVisibilities{i} = 'on';
      |    end
      | else
      |    for i=7:12
      |         MaskVisibilities{i} = 'off';
      |    end
      | end
      | set_param(gcb,'MaskVisibilities',MaskVisibilities);
      mask TypeOptions Module: 0 | 1
      mask TypeOptions SubModule: 0 | 1 | 2 | 3
      mask TypeOptions isrPriority: 0 | 1 | 2 | 3 | 4 | 5 | 6 | 7 | 8 | 9 | 10 | 11 | 12 | 13 | 14 | 15
      mask Display:
      | disp(st);
      | port_label('output',1,'trigger');
  FlexPWM ISR enable-disable : S-Function  Priority=2  FunctionName=pwm_564xl_disable_interrupt  Parameters=uint16(intSrc),uint16(subMod),uint16(pwmMod)  SFunctionDeploymentMode=off  EnableBusSupport=off  mask(PWM_564xL_disable_interrupt){intSrc=0, Module=0, pwmMod=0, SubModule=0, subMod=0, val0=off, val1=off, val2=off, val3=off, val4=off, val5=off, reload=off, reload_err=off}
      mask prompts: intSrc "int source"; pwmMod "mod"; val0 "Enable VAL0 compare interrupt"; val1 "Enable VAL1 compare interrupt"; val2 "Enable VAL2 compare interrupt"; val3 "Enable VAL3 compare interrupt"; val4 "Enable VAL4 compare interrupt"; val5 "Enable VAL5 compare interrupt"; reload "Enable Reload interrupt"; reload_err "Enable Reload error interrupt"
      mask help: FlexPWM interrupt enable/disable
      mask init:
      | Mod = get_param(gcb,'Module');
      | SubMod = get_param(gcb,'SubModule');
      | set_param(gcb,'pwmMod',num2str(Mod));
      | set_param(gcb,'subMod',num2str(SubMod));
      | crlf= sprintf('\n');
      | 
      | cmpf = 0;
      | for i = 0:5
      |     if (strcmp(get_param (gcb, ['val',num2str(i)]),'on'))
      |          cmpf = bitset(uint16(cmpf),i+1);
      |     end
      | end
      | if (strcmp(get_param (gcb, 'reload'),'on'))
      |    cmpf = bitset(uint16(cmpf),12+1);
      | end
      | if (strcmp(get_param (gcb, 'reload_err'),'on'))
      |    cmpf = bitset(uint16(cmpf),13+1);
      | end
      | set_param(gcb,'intSrc',num2str(cmpf));
      | 
      | st=['PWM Module: ',Mod,'   Sub Module: ',SubMod,crlf,'Interrupt Enable (INTEN): ',dec2bin(cmpf,16)];
      mask Help: web([rappid_block_help,filesep,'PWM_isr_enable.htm']);
      mask TypeOptions Module: 0 | 1
      mask TypeOptions SubModule: 0 | 1 | 2 | 3
      mask Display: disp(st);
  Simple PWM Output : S-Function  Priority=1  FunctionName=Simple_PWM_564xL_output  Parameters=pwmMod,subMod,uint32(InitFreq),uint16(InitDutyA),uint16(InitDutyB),centered,uint16(PhaseShift_A),uint16(PhaseShift),doubleSw,pcrNumA,pcrNumB,pcrNumX,uint16(outTrig),masterSync,debug_mode,uint16(octrl),resValue  SFunctionDeploymentMode=off  EnableBusSupport=off  mask(Simple_PWM_564xL_output){pwmModule=0, pwmMod=0, SubModule=0, subMod=0, InitFreq=0, resolution=1 %, resValue=1, InitDutyA=0, InitDutyB=0, align=A - edge aligned B - phase shifted, PhaseShift_A=0, PhaseShift=0, Phase_A=0, Phase_B=0, centered=-1, DoubleS=off, doubleSw=off, debugSw=on, debug_mode=1, pin_A0=None, pin_B0=None, pin_X0=None, pin_A1=None, pin_B1=None, pin_X1=None, pin_A2=None, pin_B2=None, pin_X2=None, pin_A3=None, pin_B3=None, pin_X3=None, pin1_A0=None, pin1_B0=None, pin1_X0=None, pin1_A1=None, pin1_B1=None, pin1_X1=None, pin1_A2=None, pin1_B2=None, pin1_X2=None, pin1_A3=None, pin1_B3=None, pin1_X3=None, pcrNumA=255, pcrNumB=255, pcrNumX=255, polA=off, polB=off, polX=off, octrl=0, syncFrom0=off, masterSync=0, outVal0=off, outVal1=off, outVal2=on, outVal3=on, outVal4=on, outVal5=on, outTrig=60}
      mask prompts: pwmModule "Module"; pwmMod "Module"; SubModule "Submodule (0-3)"; subMod "subModule (0 - 3)"; InitFreq "Initial Frequency Hz"; resValue "Resolution"; InitDutyA "PWM23: initial DutyCycle A (0..100)"; InitDutyB "PWM45: initial DutyCycle B (0..100)"; align "PWM signals"; PhaseShift_A "PWM23: initial phase shift (0..100)"; PhaseShift "PWM45: initial phase shift (0..100)"; Phase_A "PWM23 phase shift"; Phase_B "PWM45 phase shift"; centered "center aligned"; DoubleS "Double Switching"; doubleSw "double en/dis"; debugSw "Duty Cycle Simulation output"; debug_mode "Duty Cycle Simulation output"; pin_A0 "A[0] output pin"; pin_B0 "B[0] output pin"; pin_X0 "X[0] output pin"; pin_A1 "A[1] output pin"; pin_B1 "B[1] output pin"; pin_X1 "X[1] output pin"; pin_A2 "A[2] output pin"; pin_B2 "B[2] output pin"; pin_X2 "X[2] output pin"; pin_A3 "A[3] output pin"; pin_B3 "B[3] output pin"; pin_X3 "X[3] output pin"; pin1_A0 "A[0] output pin"; pin1_B0 "B[0] output pin"; pin1_X0 "X[0] output pin"; pin1_A1 "A[1] output pin"; pin1_B1 "B[1] output pin"; pin1_X1 "X[1] output pin"; pin1_A2 "A[2] output pin"; pin1_B2 "B[2] output pin"; pin1_X2 "X[2] output pin"; pin1_A3 "A[3] output pin"; pin1_B3 "B[3] output pin"; pin1_X3 "X[3] output pin"; polA "Invert PWMA Output Polarity"; polB "Invert PWMB Output Polarity"; polX "Invert PWMX Output Polarity"; syncFrom0 "Counter synchronization from Submodule 0"; masterSync "Counter synchronization"; outVal0 "VAL0"; outVal1 "VAL1"; outVal2 "VAL2"; outVal3 "VAL3"; outVal4 "VAL4"; outVal5 "VAL5"; outTrig "Output Trigger"
      mask help: Simple PWM output with frequency and duty cycle input control.
      mask init:
      | PwmMod = get_param(gcb,'pwmModule');
      | SubMod = get_param(gcb,'SubModule');
      | 
      | crlf= sprintf('\n');
      | st = [''];
      | labels = [];
      | str_disp = 'disp(st);';
      | 
      | str_pi1 = 'port_label(''input'',1,''Frequency'')';
      | str_pi2 = 'port_label(''input'',2,''Duty Cycle A'')';
      | str_pi3 = 'port_label(''input'',3,''Duty Cycle B'')';
      | str_pi4 = 'port_label(''input'',4,''Phase Shift A'')';
      | str_pi4a = 'port_label(''input'',4,''Phase Shift B'')';
      | str_pi5 = 'port_label(''input'',5,''Phase Shift B'')';
      | 
      | str_po1 = 'port_label(''output'',1,''Duty Cycle A'')';
      | str_po2 = 'port_label(''output'',2,''Duty Cycle B'')';
      | 
      | r = get_param(gcb,'resolution');
      | if isempty(strfind(r,'.001'))==0
      |   res = 1000;
      | elseif isempty(strfind(r,'.01'))==0
      |   res = 100;
      | elseif isempty(strfind(r,'.1'))==0
      |   res = 10;
      | else
      |   res = 1;
      | end
      | set_param(gcb,'resValue',num2str(res));
      | 
      | freq = num2str(get_param(gcb,'InitFreq'));
      | dutyA = num2str(str2num(get_param(gcb,'InitDutyA'))/res);
      | dutyB = num2str(str2num(get_param(gcb,'InitDutyB'))/res);
      | phaseA = num2str(str2num(get_param(gcb,'PhaseShift_A'))/res);
      | phaseB = num2str(str2num(get_param(gcb,'PhaseShift'))/res);
      | 
      | aligned = get_param(gcb,'align');
      | strA = ['PWM A init: duty cycle ',dutyA,'%'];
      | strB = ['PWM B init: duty cycle ',dutyB,'%'];
      | if strcmp(aligned,'A B - phase shifted')==1,
      |     strA = [strA,' phase shift ',phaseA,'%'];
      |     strB = [strB,' phase shift ',phaseB,'%'];
      |     set_param(gcb,'Phase_A',phaseA);
      |     set_param(gcb,'Phase_B',phaseB);
      |     labels = [labels str_pi4 char(10)];
      |     labels = [labels str_pi5 char(10)];
      |     centered = -1;    
      |     set_param(gcb,'centered','-1');
      | elseif strcmp(aligned,'A - edge aligned B - phase shifted')==1,
      |     strA = [strA,' phase shift ','0','%'];
      |     strB = [strB,' phase shift ',phaseB,'%'];
      |     set_param(gcb,'Phase_A','0');
      |     set_param(gcb,'Phase_B',phaseB);
      |     labels = [labels str_pi4a char(10)];
      |     centered = -2;    
      |     set_param(gcb,'centered','-1');
      | else
      |     set_param(gcb,'Phase_A','0');
      |     set_param(gcb,'Phase_B','0');
      |     if strcmp(aligned,'A B - center aligned')==1,
      |         centered = 1;    
      |         set_param(gcb,'centered','1');
      |         strA = [strA,' center aligned'];
      |         strB = [strB,' center aligned'];
      |     else
      |         centered = 0;    
      |         set_param(gcb,'centered','0');
      |         strA = [strA,' edge aligned'];
      |         strB = [strB,' edge aligned'];
      |     end
      | end
      | 
      | if strcmp(get_param(gcb,'DoubleS'),'on')==1,
      |    dbl = 'Double switching Enabled';
      |    doubleSw = 1;
      | else
      |    dbl = 'Double switching Disabled';
      |    doubleSw = 0;
      | end    
      | 
      | if strcmp(get_param(gcb,'debugSw'),'on')==1,
      |    debug_mode = 1;   
      |    set_param(gcb,'debug_mode','1');
      |    labels = [labels str_po1 char(10)];
      |    labels = [labels str_po2 char(10)];
      | else
      |    debug_mode = 0;   
      |    set_param(gcb,'debug_mode','0');
      | end
      | 
      | mod = num2str(SubMod);
      | set_param(gcb,'subMod',mod);
      | 
      | pwm_m = num2str(PwmMod);
      | set_param(gcb,'pwmMod',pwm_m);
      | if strcmp(pwm_m,'0')==0
      |     pwmStr = pwm_m;
      | else
      |     pwmStr = '';
      | end
      | 
      | pcrStr = get_param(gcb,['pin',pwmStr,'_A',mod]);
      | if strcmp(pcrStr,'None')==1
      |    set_param(gcb,'pcrNumA','255');
      | else    
      |    posColon = findstr(pcrStr, ':');
      |    num = strtrim(pcrStr(1:posColon(1)-1));
      |    set_param(gcb,'pcrNumA',num);
      | end
      | 
      | pcrStr = get_param(gcb,['pin',pwmStr,'_B',mod]);
      | if strcmp(pcrStr,'None')==1
      |    set_param(gcb,'pcrNumB','255');
      | else    
      |    posColon = findstr(pcrStr, ':');
      |    num = strtrim(pcrStr(1:posColon(1)-1));
      |    set_param(gcb,'pcrNumB',num);
      | end
      | 
      | pcrStr = get_param(gcb,['pin',pwmStr,'_X',mod]);
      | if strcmp(pcrStr,'None')==1
      |    set_param(gcb,'pcrNumX','255');
      | else    
      |    posColon = findstr(pcrStr, ':');
      |    num = strtrim(pcrStr(1:posColon(1)-1));
      |    set_param(gcb,'pcrNumX',num);
      | end
      | 
      | st= ['PWM Module: ',PwmMod,'   Sub Module: ',SubMod, ...
      |     crlf,'Initial Frequency  ',freq,'Hz',crlf, ...
      |     strA,crlf,strB,crlf,dbl];
      | 
      | labels = [labels str_disp char(10)];
      | labels = [labels str_pi1 char(10)];
      | labels = [labels str_pi2 char(10)];
      | labels = [labels str_pi3 char(10)];
      | 
      | labels(end) = [];
      | set_param(gcb,'MaskDisplay',labels);
      | 
      | outT = 0;
      | for i = 0:5
      |     if (strcmp(get_param (gcb, ['outVal',num2str(i)]),'on'))
      |          outT = bitset(uint16(outT),i+1);
      |     end
      | end
      | set_param(gcb,'outTrig',num2str(outT));
      | 
      | if strcmp(get_param(gcb,'syncFrom0'),'on')==1,
      |    set_param(gcb,'masterSync','1');
      | else
      |    set_param(gcb,'masterSync','0');
      | end
      | 
      | polarityABX = 0;
      | if strcmp(get_param(gcb,'polA'),'on')==1,
      |    polarityABX = bitset(uint16(polarityABX),11);
      | end
      | if strcmp(get_param(gcb,'polB'),'on')==1,
      |    polarityABX = bitset(uint16(polarityABX),10);
      | end
      | if strcmp(get_param(gcb,'polX'),'on')==1,
      |    polarityABX = bitset(uint16(polarityABX),9);
      | end
      | set_param(gcb,'octrl',num2str(polarityABX));
      mask Help: web([rappid_block_help,filesep,'Simple_PWM_output.htm']);
      mask TypeOptions pwmModule: 0 | 1
      mask Callback pwmModule: rappid_564xl_block_pwm_change_mod (gcb, 20,3,51);
      mask TypeOptions SubModule: 0 | 1 | 2 | 3
      mask Callback SubModule: rappid_564xl_block_pwm_change_mod (gcb,20,3,51);
      mask TypeOptions resolution: 1 % | 0.1 % | 0.01 % | 0.001 %
      mask Callback resolution:
      | MaskPrompts = get_param(gcb,'MaskPrompts');
      | r = get_param(gcb,'resolution');
      | if isempty(strfind(r,'.001'))==0
      |   mStr = regexprep(MaskPrompts{8},'..\d+\)','..100000)');
      |   if strcmp(mStr,MaskPrompts{8})==0
      |      MaskPrompts{8} = regexprep(MaskPrompts{8},'..\d+\)','..100000)');
      |      MaskPrompts{9} = regexprep(MaskPrompts{9},'..\d+\)','..100000)');
      |      MaskPrompts{11} = regexprep(MaskPrompts{11},'..\d+\)','..100000)');
      |      MaskPrompts{12} = regexprep(MaskPrompts{12},'..\d+\)','..100000)');
      |      set_param(gcb,'MaskPrompts',MaskPrompts);
      |   end
      | elseif isempty(strfind(r,'.01'))==0
      |   mStr = regexprep(MaskPrompts{8},'..\d+\)','..10000)');
      |   if strcmp(mStr,MaskPrompts{8})==0
      |      MaskPrompts{8} = regexprep(MaskPrompts{8},'..\d+\)','..10000)');
      |      MaskPrompts{9} = regexprep(MaskPrompts{9},'..\d+\)','..10000)');
      |      MaskPrompts{11} = regexprep(MaskPrompts{11},'..\d+\)','..10000)');
      |      MaskPrompts{12} = regexprep(MaskPrompts{12},'..\d+\)','..10000)');
      |      set_param(gcb,'MaskPrompts',MaskPrompts);
      |   end
      | elseif isempty(strfind(r,'.1'))==0
      |   mStr = regexprep(MaskPrompts{8},'..\d+\)','..1000)');
      |   if strcmp(mStr,MaskPrompts{8})==0
      |      MaskPrompts{8} = regexprep(MaskPrompts{8},'..\d+\)','..1000)');
      |      MaskPrompts{9} = regexprep(MaskPrompts{9},'..\d+\)','..1000)');
      |      MaskPrompts{11} = regexprep(MaskPrompts{11},'..\d+\)','..1000)');
      |      MaskPrompts{12} = regexprep(MaskPrompts{12},'..\d+\)','..1000)');
      |      set_param(gcb,'MaskPrompts',MaskPrompts);
      |   end
      | else
      |   mStr = regexprep(MaskPrompts{8},'..\d+\)','..100)');
      |   if strcmp(mStr,MaskPrompts{8})==0
      |      MaskPrompts{8} = regexprep(MaskPrompts{8},'..\d+\)','..100)');
      |      MaskPrompts{9} = regexprep(MaskPrompts{9},'..\d+\)','..100)');
      |      MaskPrompts{11} = regexprep(MaskPrompts{11},'..\d+\)','..100)');
      |      MaskPrompts{12} = regexprep(MaskPrompts{12},'..\d+\)','..100)');
      |      set_param(gcb,'MaskPrompts',MaskPrompts);
      |   end
      | end
      mask TypeOptions align: A - edge aligned B - phase shifted | A B - center aligned | A B - edge aligned | A B - phase shifted
      mask Callback align:
      | MaskVisibilities = get_param(gcb,'MaskVisibilities');
      | if strcmp(get_param(gcb,'align'),'A B - phase shifted')==1,
      |     MaskVisibilities{11} = 'on';
      |     MaskVisibilities{12} = 'on';
      | elseif strcmp(get_param(gcb,'align'),'A - edge aligned B - phase shifted')==1,
      |     MaskVisibilities{11} = 'off';
      |     MaskVisibilities{12} = 'on';
      | else
      |     MaskVisibilities{11} = 'off';
      |     MaskVisibilities{12} = 'off';
      | end
      | set_param(gcb,'MaskVisibilities',MaskVisibilities);
      mask TypeOptions pin_A0: None | 11  : PA11 : [ 120 ] : [ D11 ] | 58  : PD10 : [ 76 ] : [ T15 ]
      mask TypeOptions pin_B0: None | 10  : PA10 : [ 118 ] : [A13 ] | 59  : PD11 : [ 78 ] : [ R16 ]
      mask TypeOptions pin_X0: None | 57  : PD9 : [ 26 ] : [ L3 ]
      mask TypeOptions pin_A1: None | 39  : PC7  : [ 15 ] : [ K4 ] | 47  : PC15 : [ 124 ] : [ A8 ] | 80  : PF0  : [ 133 ] : [ D7 ]
      mask TypeOptions pin_B1: None | 38  : PC6  : [ 142 ] : [ D4 ] | 48  : PD0  : [ 125 ] : [ B8 ] | 62  : PD14 : [ 105 ] : [ D16 ]
      mask TypeOptions pin_X1: None | 36  : PC4 : [ 11 ] : [ H3 ] | 60  : PD12 : [ 99 ] : [ G14 ]
      mask TypeOptions pin_A2: None | 11  : PA11 : [ 120 ] : [ D11 ] | 12  : PA12 : [ 122 ] : [ A10 ] | 99  : PG3  : [ 104 ] : [ D17 ]
      mask TypeOptions pin_B2: None | 12  : PA12 : [ 122 ] : [ A10 ] | 13  : PA13 : [ 136 ] : [ C6 ] | 100 : PG4  : [ 100 ] : [ F17 ]
      mask TypeOptions pin_X2: None | 10  : PA10 : [ 118 ] : [A13 ] | 98  : PG2 : [ 102 ] : [ E16 ]
      mask TypeOptions pin_A3: None | 2   : PA2  : [ 84 ] : [ N16 ] | 42  : PC10 : [ 111 ] : [ A15 ] | 51  : PD3  : [ 128 ] : [ A7 ] | 102 : PG6  : [ 98 ] : [ G17 ]
      mask TypeOptions pin_B3: None | 3   : PA3  : [ 92 ] : [ K17 ] | 9   : PA9  : [ 134 ] : [ B6 ] | 52  : PD4  : [ 129 ] : [ B7 ] | 103 : PG7  : [ 83 ] : [ P17 ]
      mask TypeOptions pin_X3: None | 50  : PD2 : [ 140 ] : [ C5 ] | 54  : PD6 : [ 34 ] : [ P3 ] | 101  : PG5 : [ 85 ] : [ N17 ]
      mask TypeOptions pin1_A0: None | 117 : PH5 : [ --- ] : [ M17 ]
      mask TypeOptions pin1_B0: None | 118 : PH6 : [ --- ] : [ H17 ]
      mask TypeOptions pin1_X0: None | 116 : PH4 : [ --- ] : [ L16 ]
      mask TypeOptions pin1_A1: None | 120 : PH8 : [ --- ] : [ K15 ]
      mask TypeOptions pin1_B1: None | 121 : PH9 : [ --- ] : [ G16 ]
      mask TypeOptions pin1_X1: None | 119 : PH7 : [ --- ] : [ K16 ]
      mask TypeOptions pin1_A2: None | 123 : PH11 : [ --- ] : [ C11 ]
      mask TypeOptions pin1_B2: None | 124 : PH12 : [ --- ] : [ B10 ]
      mask TypeOptions pin1_X2: None | 122 : PH10 : [ --- ] : [ A11 ]
      mask TypeOptions pin1_A3: None | 126 : PH14 : [ --- ] : [ A12 ]
      mask TypeOptions pin1_B3: None | 127 : PH15 : [ --- ] : [ J17 ]
      mask TypeOptions pin1_X3: None | 125 : PH13 : [ --- ] : [ G15 ]
      mask Display:
      | port_label('input',4,'Phase Shift B')
      | port_label('output',1,'Duty Cycle A')
      | port_label('output',2,'Duty Cycle B')
      | disp(st);
      | port_label('input',1,'Frequency')
      | port_label('input',2,'Duty Cycle A')
      | port_label('input',3,'Duty Cycle B')
  Sine Wave Generator : S-Function  FunctionName=sineWave_564xl  Parameters=uint16(frequency),uint8(IOAMPL)  SFunctionDeploymentMode=off  EnableBusSupport=off  mask(sineWave_564xL){amplitude=0.467, frequency=2000, IOAMPL=0}
      mask prompts: amplitude "Amplitude, V"; frequency "Frequency, Hz (1000 - 50000)"
      mask help: Sine Wave Generator
      mask init:
      | amplitude = get_param(gcb,'amplitude');
      | freq = get_param(gcb,'frequency');
      | 
      | if strcmp(amplitude,'0.467')==1
      |     set_param(gcb,'IOAMPL','0');
      | elseif strcmp(amplitude,'0.538')==1
      |     set_param(gcb,'IOAMPL','1');
      | elseif strcmp(amplitude,'0.611')==1
      |     set_param(gcb,'IOAMPL','2');
      | elseif strcmp(amplitude,'0.682')==1
      |     set_param(gcb,'IOAMPL','3');
      | elseif strcmp(amplitude,'0.754')==1
      |     set_param(gcb,'IOAMPL','4');
      | elseif strcmp(amplitude,'0.826')==1
      |     set_param(gcb,'IOAMPL','5');
      | elseif strcmp(amplitude,'0.898')==1
      |     set_param(gcb,'IOAMPL','6');
      | elseif strcmp(amplitude,'0.969')==1
      |     set_param(gcb,'IOAMPL','7');
      | elseif strcmp(amplitude,'1.090')==1
      |     set_param(gcb,'IOAMPL','8');
      | elseif strcmp(amplitude,'1.258')==1
      |     set_param(gcb,'IOAMPL','9');
      | elseif strcmp(amplitude,'1.426')==1
      |     set_param(gcb,'IOAMPL','10');
      | elseif strcmp(amplitude,'1.595')==1
      |     set_param(gcb,'IOAMPL','11');
      | elseif strcmp(amplitude,'1.761')==1
      |     set_param(gcb,'IOAMPL','12');
      | elseif strcmp(amplitude,'1.929')==1
      |     set_param(gcb,'IOAMPL','13');
      | elseif strcmp(amplitude,'2.097')==1
      |     set_param(gcb,'IOAMPL','14');
      | else
      |     set_param(gcb,'IOAMPL','15');
      | end    
      |     
      | crlf= sprintf('\n');
      | st=['Amplitude ',amplitude ,' V',crlf,'Frequency ',freq,' Hz'];
      mask Help: web([rappid_block_help,filesep,'sine_wave_generator.htm']);
      mask TypeOptions amplitude: 0.467 | 0.538 | 0.611 | 0.682 | 0.754 | 0.826 | 0.898 | 0.969 | 1.090 | 1.258 | 1.426 | 1.595 | 1.761 | 1.929 | 2.097 | 2.264
      mask Display:
      | disp(st);
      | port_label('input',1,'Frequency')
  Three Phase PWM Output : S-Function  FunctionName=ThreePhase_PWM_564xL_output  Parameters=pwmMod,subMod,uint32(InitFreq),uint16(InitDutyA),uint16(InitDutyB),uint16(InitDutyC),uint16(DeadTime),pcrNum,outTrig,debug_mode,deadtime_mks,octrl,resValue  SFunctionDeploymentMode=off  EnableBusSupport=off  mask(ThreePhase_PWM_564xL_output){pwmModule=0, pwmMod=0, SubModule=0 1 2, subMod=0, InitFreq=0, resolution=1 %, resValue=1, InitDutyA=0, InitDutyB=0, InitDutyC=0, DeadTime=0, dt=IPBus clock cycles, deadtime_mks=0, DebugSw=on, debug_mode=1, pin_A0=None, pin_B0=None, pin_A1=None, pin_B1=None, pin_A2=None, pin_B2=None, pin_A3=None, pin_B3=None, pin1_A0=None, pin1_B0=None, pin1_A1=None, pin1_B1=None, pin1_A2=None, pin1_B2=None, pin1_A3=None, pin1_B3=None, pcrNum=0, polA0=off, polB0=off, polA1=off, polB1=off, polA2=off, polB2=off, polA3=off, polB3=off, octrl=0, outVal_A0=off, outVal_A1=off, outVal_A2=on, outVal_A3=on, outVal_B0=off, outVal_B1=off, outVal_B2=on, outVal_B3=on, outVal_C0=off, outVal_C1=off, outVal_C2=on, outVal_C3=on, outTrig=0}
      mask prompts: pwmModule "Module"; pwmMod "Module"; SubModule "Submodules A B C"; subMod "subModule (0 - 3)"; InitFreq "Initial Frequency, Hz"; resValue "Resolution"; InitDutyA "Initial DutyCycle A (0..100)"; InitDutyB "Initial DutyCycle B (0..100)"; InitDutyC "Initial DutyCycle C (0..100)"; DeadTime "Initial Deadtime"; dt "Deadtime values in"; DebugSw "Duty Cycle Simulation Output"; debug_mode "Duty Cycle Simulation Output"; pin_A0 "A[0] output pin"; pin_B0 "B[0] output pin"; pin_A1 "A[1] output pin"; pin_B1 "B[1] output pin"; pin_A2 "A[2] output pin"; pin_B2 "B[2] output pin"; pin_A3 "A[3] output pin"; pin_B3 "B[3] output pin"; pin1_A0 "A[0] output pin"; pin1_B0 "B[0] output pin"; pin1_A1 "A[1] output pin"; pin1_B1 "B[1] output pin"; pin1_A2 "A[2] output pin"; pin1_B2 "B[2] output pin"; pin1_A3 "A[3] output pin"; pin1_B3 "B[3] output pin"; polA0 "Invert PWMA[0] Output Polarity"; polB0 "Invert PWMB[0] Output Polarity"; polA1 "Invert PWMA[1] Output Polarity"; polB1 "Invert PWMB[1] Output Polarity"; polA2 "Invert PWMA[2] Output Polarity"; polB2 "Invert PWMB[2] Output Polarity"; polA3 "Invert PWMA[3] Output Polarity"; polB3 "Invert PWMB[3] Output Polarity"; outVal_A0 "PWM A VAL0"; outVal_A1 "PWM A VAL1"; outVal_A2 "PWM A VAL2"; outVal_A3 "PWM A VAL3"; outVal_B0 "PWM B VAL0"; outVal_B1 "PWM B VAL1"; outVal_B2 "PWM B VAL2"; outVal_B3 "PWM B VAL3"; outVal_C0 "PWM C VAL0"; outVal_C1 "PWM C VAL1"; outVal_C2 "PWM C VAL2"; outVal_C3 "PWM C VAL3"; outTrig "Output Trigger"
      mask help: Three-phase PWM output with deadtime insertion with frequency and duty cycle input control.
      mask init:
      | PwmMod = get_param(gcb,'pwmModule');
      | SubMod = get_param(gcb,'SubModule');
      | crlf= sprintf('\n');
      | st = [''];
      | labels = [];
      | str_disp = 'disp(st);';
      | 
      | str_pi1 = 'port_label(''input'',1,''Frequency'')';
      | str_pi2 = 'port_label(''input'',2,''Duty Cycle A'')';
      | str_pi3 = 'port_label(''input'',3,''Duty Cycle B'')';
      | str_pi4 = 'port_label(''input'',4,''Duty Cycle C'')';
      | str_pi5 = 'port_label(''input'',5,''PWMA Deadtime'')';
      | str_pi6 = 'port_label(''input'',6,''PWMB Deadtime'')';
      | 
      | str_po1 = 'port_label(''output'',1,''Duty Cycle A'')';
      | str_po2 = 'port_label(''output'',2,''Duty Cycle B'')';
      | str_po3 = 'port_label(''output'',3,''Duty Cycle C'')';
      | 
      | r = get_param(gcb,'resolution');
      | if isempty(strfind(r,'.001'))==0
      |   res = 1000;
      | elseif isempty(strfind(r,'.01'))==0
      |   res = 100;
      | elseif isempty(strfind(r,'.1'))==0
      |   res = 10;
      | else
      |   res = 1;
      | end
      | set_param(gcb,'resValue',num2str(res));
      | 
      | freq = num2str(get_param(gcb,'InitFreq'));
      | dutyA = num2str(str2num(get_param(gcb,'InitDutyA'))/res);
      | dutyB = num2str(str2num(get_param(gcb,'InitDutyB'))/res);
      | dutyC = num2str(str2num(get_param(gcb,'InitDutyC'))/res);
      | dt = num2str(get_param(gcb,'DeadTime'));
      | 
      | if strcmp(get_param(gcb,'dt'),'microseconds')==1,
      |    set_param(gcb,'deadtime_mks','1');
      |    dt_str = ' microseconds';
      | else
      |    set_param(gcb,'deadtime_mks','0');
      |    dt_str = ' IPBus cycles';
      | end
      | 
      | pwm_m = num2str(PwmMod);
      | set_param(gcb,'pwmMod',pwm_m);
      | if strcmp(pwm_m,'0')==0
      |     pwmStr = pwm_m;
      | else
      |     pwmStr = '';
      | end
      | 
      | st=['PWM Module: ',PwmMod,'   Sub Modules ',SubMod,crlf,' Initial Frequency  ',freq,'Hz',crlf,...
      |     ' Initial DutyCycle A ',dutyA,'% ',crlf,' Initial DutyCycle B ',dutyB,'% ',crlf,...
      |     ' Initial DutyCycle C ',dutyC,'% ',crlf,' Initial DeadTime ',dt,dt_str];
      | 
      | if strcmp(get_param(gcb,'debugSw'),'on')==1,
      |    debug_mode = 1;
      |    set_param(gcb,'debug_mode','1');
      |    labels = [labels str_po1 char(10)];
      |    labels = [labels str_po2 char(10)];
      |    labels = [labels str_po3 char(10)];   
      | else
      |    debug_mode = 0;
      |    set_param(gcb,'debug_mode','0');
      | end
      | 
      | labels = [labels str_disp char(10)];
      | labels = [labels str_pi1 char(10)];
      | labels = [labels str_pi2 char(10)];
      | labels = [labels str_pi3 char(10)];
      | labels = [labels str_pi4 char(10)];
      | labels = [labels str_pi5 char(10)];
      | labels = [labels str_pi6 char(10)];
      | 
      | labels(end) = [];
      | set_param(gcb,'MaskDisplay',labels);
      | 
      | pcrNum = [255, 255, 255, 255, 255, 255];
      | octrl = [0, 0, 0];
      | 
      | if strcmp(SubMod,'0 1 2')==1,
      |     set_param(gcb,'subMod','0');
      | elseif  strcmp(SubMod,'0 1 3')==1,
      |     set_param(gcb,'subMod','1');
      | elseif  strcmp(SubMod,'0 2 3')==1,
      |     set_param(gcb,'subMod','2');
      | end
      | 
      |   pcrStr = get_param(gcb,['pin',pwmStr,'_A0']);
      |   if strcmp(pcrStr,'None')==1
      |      pcrNumArr{1} = 255;     
      |   else    
      |      posColon = findstr(pcrStr, ':');
      |      num = strtrim(pcrStr(1:posColon(1)-1));
      |      pcrNumArr{1} = str2num(num);     
      |   end
      |   pcrStr = get_param(gcb,['pin',pwmStr,'_B0']);
      |   if strcmp(pcrStr,'None')==1
      |      pcrNumArr{2} = 255;     
      |   else    
      |      posColon = findstr(pcrStr, ':');
      |      num = strtrim(pcrStr(1:posColon(1)-1));
      |      pcrNumArr{2} = str2num(num);     
      |   end
      |   pcrInd = 3;
      |   polarityAB = 0;
      |   if strcmp(get_param(gcb,'polA0'),'on')==1,
      |     polarityAB = bitset(uint16(polarityAB),11);
      |   end
      |   if strcmp(get_param(gcb,'polB0'),'on')==1,
      |     polarityAB = bitset(uint16(polarityAB),10);
      |   end
      |   polarityArr{1} = polarityAB;
      |   polInd = 2;
      | 
      | if  strcmp(SubMod,'0 2 3')==0
      |   pcrStr = get_param(gcb,['pin',pwmStr,'_A1']);
      |   if strcmp(pcrStr,'None')==1
      |      pcrNumArr{3} = 255;     
      |   else    
      |      posColon = findstr(pcrStr, ':');
      |      num = strtrim(pcrStr(1:posColon(1)-1));
      |      pcrNumArr{3} = str2num(num);     
      |   end
      |   pcrStr = get_param(gcb,['pin',pwmStr,'_B1']);
      |   if strcmp(pcrStr,'None')==1
      |      pcrNumArr{4} = 255;     
      |   else    
      |      posColon = findstr(pcrStr, ':');
      |      num = strtrim(pcrStr(1:posColon(1)-1));
      |      pcrNumArr{4} = str2num(num);     
      |   end
      |   pcrInd = 5;
      |   polarityAB = 0;
      |   if strcmp(get_param(gcb,'polA1'),'on')==1,
      |     polarityAB = bitset(uint16(polarityAB),11);
      |   end
      |   if strcmp(get_param(gcb,'polB1'),'on')==1,
      |     polarityAB = bitset(uint16(polarityAB),10);
      |   end
      |   polarityArr{2} = polarityAB;
      |   polInd = 3;
      | end
      | 
      | if  strcmp(SubMod,'0 1 3')==0
      |   pcrStr = get_param(gcb,['pin',pwmStr,'_A2']);
      |   if strcmp(pcrStr,'None')==1
      |     pcrNumArr{pcrInd} = 255;     
      |   else    
      |      posColon = findstr(pcrStr, ':');
      |      num = strtrim(pcrStr(1:posColon(1)-1));
      |      pcrNumArr{pcrInd} = str2num(num);     
      |   end
      |   pcrStr = get_param(gcb,['pin',pwmStr,'_B2']);
      |   if strcmp(pcrStr,'None')==1
      |      pcrNumArr{pcrInd+1} = 255;     
      |   else    
      |      posColon = findstr(pcrStr, ':');
      |      num = strtrim(pcrStr(1:posColon(1)-1));
      |      pcrNumArr{pcrInd+1} = str2num(num);     
      |   end
      |   polarityAB = 0;
      |   if strcmp(get_param(gcb,'polA2'),'on')==1,
      |     polarityAB = bitset(uint16(polarityAB),11);
      |   end
      |   if strcmp(get_param(gcb,'polB2'),'on')==1,
      |     polarityAB = bitset(uint16(polarityAB),10);
      |   end
      |   polarityArr{polInd} = polarityAB;
      | end
      |     
      | if strcmp(SubMod,'0 1 2')==0
      |   pcrStr = get_param(gcb,['pin',pwmStr,'_A3']);
      |   if strcmp(pcrStr,'None')==1
      |      pcrNumArr{5} = 255;     
      |   else    
      |      posColon = findstr(pcrStr, ':');
      |      num = strtrim(pcrStr(1:posColon(1)-1));
      |      pcrNumArr{5} = str2num(num);     
      |   end
      |   pcrStr = get_param(gcb,['pin',pwmStr,'_B3']);
      |   if strcmp(pcrStr,'None')==1
      |      pcrNumArr{6} = 255;     
      |   else    
      |      posColon = findstr(pcrStr, ':');
      |      num = strtrim(pcrStr(1:posColon(1)-1));
      |      pcrNumArr{6} = str2num(num);     
      |   end
      |   polarityAB = 0;
      |   if strcmp(get_param(gcb,'polA3'),'on')==1,
      |     polarityAB = bitset(uint16(polarityAB),11);
      |   end
      |   if strcmp(get_param(gcb,'polB3'),'on')==1,
      |     polarityAB = bitset(uint16(polarityAB),10);
      |   end
      |   polarityArr{3} = polarityAB;
      | end
      | 
      | pcrNum = [pcrNumArr{1},pcrNumArr{2},pcrNumArr{3},pcrNumArr{4},pcrNumArr{5},pcrNumArr{6}];
      | octrl = [polarityArr{1},polarityArr{2},polarityArr{3}];
      | 
      | outT_A = 0;
      | outT_B = 0;
      | outT_C = 0;
      | for i = 0:3
      |     if (strcmp(get_param (gcb, ['outVal_A',num2str(i)]),'on'))
      |          outT_A = bitset(uint16(outT_A),i+1);
      |     end
      |     if (strcmp(get_param (gcb, ['outVal_B',num2str(i)]),'on'))
      |          outT_B = bitset(uint16(outT_B),i+1);
      |     end
      |     if (strcmp(get_param (gcb, ['outVal_C',num2str(i)]),'on'))
      |          outT_C = bitset(uint16(outT_C),i+1);
      |     end
      | end
      | outTrig = [outT_A, outT_B, outT_C];
      mask Help: web([rappid_block_help,filesep,'ThreePhase_PWM_output.htm']);
      mask TypeOptions pwmModule: 0 | 1
      mask Callback pwmModule: rappid_564xl_block_pwm3_change_mod (gcb);
      mask TypeOptions SubModule: 0 1 2 | 0 1 3 | 0 2 3
      mask Callback SubModule: rappid_564xl_block_pwm3_change_mod (gcb);
      mask TypeOptions resolution: 1 % | 0.1 % | 0.01 % | 0.001 %
      mask Callback resolution:
      | MaskPrompts = get_param(gcb,'MaskPrompts');
      | r = get_param(gcb,'resolution');
      | if isempty(strfind(r,'.001'))==0
      |   mStr = regexprep(MaskPrompts{8},'..\d+\)','..100000)');
      |   if strcmp(mStr,MaskPrompts{8})==0
      |      MaskPrompts{8} = regexprep(MaskPrompts{8},'..\d+\)','..100000)');
      |      MaskPrompts{9} = regexprep(MaskPrompts{9},'..\d+\)','..100000)');
      |      MaskPrompts{10} = regexprep(MaskPrompts{10},'..\d+\)','..100000)');
      |      set_param(gcb,'MaskPrompts',MaskPrompts);
      |   end
      | elseif isempty(strfind(r,'.01'))==0
      |   mStr = regexprep(MaskPrompts{8},'..\d+\)','..10000)');
      |   if strcmp(mStr,MaskPrompts{8})==0
      |      MaskPrompts{8} = regexprep(MaskPrompts{8},'..\d+\)','..10000)');
      |      MaskPrompts{9} = regexprep(MaskPrompts{9},'..\d+\)','..10000)');
      |      MaskPrompts{10} = regexprep(MaskPrompts{10},'..\d+\)','..10000)');
      |      set_param(gcb,'MaskPrompts',MaskPrompts);
      |   end
      | elseif isempty(strfind(r,'.1'))==0
      |   mStr = regexprep(MaskPrompts{8},'..\d+\)','..1000)');
      |   if strcmp(mStr,MaskPrompts{8})==0
      |      MaskPrompts{8} = regexprep(MaskPrompts{8},'..\d+\)','..1000)');
      |      MaskPrompts{9} = regexprep(MaskPrompts{9},'..\d+\)','..1000)');
      |      MaskPrompts{10} = regexprep(MaskPrompts{10},'..\d+\)','..1000)');
      |      set_param(gcb,'MaskPrompts',MaskPrompts);
      |   end
      | else
      |   mStr = regexprep(MaskPrompts{8},'..\d+\)','..100)');
      |   if strcmp(mStr,MaskPrompts{8})==0
      |      MaskPrompts{8} = regexprep(MaskPrompts{8},'..\d+\)','..100)');
      |      MaskPrompts{9} = regexprep(MaskPrompts{9},'..\d+\)','..100)');
      |      MaskPrompts{10} = regexprep(MaskPrompts{10},'..\d+\)','..100)');
      |      set_param(gcb,'MaskPrompts',MaskPrompts);
      |   end
      | end
      mask TypeOptions dt: IPBus clock cycles | microseconds
      mask TypeOptions pin_A0: None | 11  : PA11 : [ 120 ] : [ D11 ] | 58  : PD10 : [ 76 ] : [ T15 ]
      mask TypeOptions pin_B0: None | 10  : PA10 : [ 118 ] : [A13 ] | 59  : PD11 : [ 78 ] : [ R16 ]
      mask TypeOptions pin_A1: None | 39  : PC7  : [ 15 ] : [ K4 ] | 47  : PC15 : [ 124 ] : [ A8 ] | 80  : PF0  : [ 133 ] : [ D7 ]
      mask TypeOptions pin_B1: None | 38  : PC6  : [ 142 ] : [ D4 ] | 48  : PD0  : [ 125 ] : [ B8 ] | 62  : PD14 : [ 105 ] : [ D16 ]
      mask TypeOptions pin_A2: None | 11  : PA11 : [ 120 ] : [ D11 ] | 12  : PA12 : [ 122 ] : [ A10 ] | 99  : PG3  : [ 104 ] : [ D17 ]
      mask TypeOptions pin_B2: None | 12  : PA12 : [ 122 ] : [ A10 ] | 13  : PA13 : [ 136 ] : [ C6 ] | 100 : PG4  : [ 100 ] : [ F17 ]
      mask TypeOptions pin_A3: None | 2   : PA2  : [ 84 ] : [ N16 ] | 42  : PC10 : [ 111 ] : [ A15 ] | 51  : PD3  : [ 128 ] : [ A7 ] | 102 : PG6  : [ 98 ] : [ G17 ]
      mask TypeOptions pin_B3: None | 3   : PA3  : [ 92 ] : [ K17 ] | 9   : PA9  : [ 134 ] : [ B6 ] | 52  : PD4  : [ 129 ] : [ B7 ] | 103 : PG7  : [ 83 ] : [ P17 ]
      mask TypeOptions pin1_A0: None | 117 : PH5 : [ --- ] : [ M17 ]
      mask TypeOptions pin1_B0: None | 118 : PH6 : [ --- ] : [ H17 ]
      mask TypeOptions pin1_A1: None | 120 : PH8 : [ --- ] : [ K15 ]
      mask TypeOptions pin1_B1: None | 121 : PH9 : [ --- ] : [ G16 ]
      mask TypeOptions pin1_A2: None | 123 : PH11 : [ --- ] : [ C11 ]
      mask TypeOptions pin1_B2: None | 124 : PH12 : [ --- ] : [ B10 ]
      mask TypeOptions pin1_A3: None | 126 : PH14 : [ --- ] : [ A12 ]
      mask TypeOptions pin1_B3: None | 127 : PH15 : [ --- ] : [ J17 ]
      mask Display:
      | port_label('output',1,'Duty Cycle A')
      | port_label('output',2,'Duty Cycle B')
      | port_label('output',3,'Duty Cycle C')
      | disp(st);
      | port_label('input',1,'Frequency')
      | port_label('input',2,'Duty Cycle A')
      | port_label('input',3,'Duty Cycle B')
      | port_label('input',4,'Duty Cycle C')
      | port_label('input',5,'PWMA Deadtime')
      | port_label('input',6,'PWMB Deadtime')
  eTimer CNTR Register Read : S-Function  FunctionName=eTimer_564xL_cntr  Parameters=uint16(subMod),uint16(channel)  SFunctionDeploymentMode=off  EnableBusSupport=off  mask(eTimer_564xL_Cntr){SubModule=0, TimerChan=0, subMod=0, channel=0}
      mask prompts: TimerChan "Channel"
      mask help: This block provides a direct read from eTimer Counter register.
      mask init:
      | SubMod = get_param(gcb,'SubModule');
      | Chan = get_param(gcb,'TimerChan');
      | 
      | set_param(gcb,'subMod',num2str(SubMod));
      | set_param(gcb,'channel',num2str(Chan));
      | 
      | crlf= sprintf('\n');
      | st=['Sub Module ',SubMod ,' Channel ',Chan];
      mask Help: web([rappid_block_help,filesep,'eTimer_cntr.htm']);
      mask TypeOptions SubModule: 0 | 1 | 2
      mask TypeOptions TimerChan: 0 | 1 | 2 | 3 | 4 | 5
      mask Display:
      | port_label('output',1,'CNTR');
      | disp(st);
  eTimer HOLD Register Read : S-Function  FunctionName=eTimer_564xL_hold  Parameters=uint16(subMod),uint16(channel)  SFunctionDeploymentMode=off  EnableBusSupport=off  mask(eTimer_564xL_Hold){SubModule=0, TimerChan=0, subMod=0, channel=0}
      mask prompts: TimerChan "Channel"
      mask help: This block provides a direct read from eTimer Hold register.
      mask init: same as rappid_564xl_ec_toolbox/MPC564xL/Motor Control Blocks/eTimer CNTR Register Read
      mask Help: web([rappid_block_help,filesep,'eTimer_hold.htm']);
      mask TypeOptions SubModule: 0 | 1 | 2
      mask TypeOptions TimerChan: 0 | 1 | 2 | 3 | 4 | 5
      mask Display:
      | port_label('output',1,'HOLD');
      | disp(st);
  eTimer ISR : S-Function  FunctionName=eTimer_564xl_interrupt  Parameters=uint16(subMod),uint16(channel),uint16(isrPrio)  SFunctionDeploymentMode=off  EnableBusSupport=off  mask(eTimer_564xL_interrupt){SubModule=0, Timerchan=0, subMod=0, channel=0, isrPriority=0, isrPrio=0}
      mask prompts: Timerchan "Channel"; isrPriority "Priority"; isrPrio "priority"
      mask help: eTimer interrupt
      mask init:
      | SubMod = get_param(gcb,'SubModule');
      | Chan = get_param(gcb,'TimerChan');
      | isrPr = get_param(gcb,'isrPriority');
      | 
      | set_param(gcb,'subMod',num2str(SubMod));
      | set_param(gcb,'channel',num2str(Chan));
      | set_param(gcb,'isrPrio',num2str(isrPr));
      | 
      | crlf= sprintf('\n');
      | st=['Sub Module ',SubMod ,' Channel ',Chan,crlf,'ISR priority: ',isrPr];
      mask Help: web([rappid_block_help,filesep,'eTimer_interrupt.htm']);
      mask TypeOptions SubModule: 0 | 1 | 2
      mask TypeOptions Timerchan: 0 | 1 | 2 | 3 | 4 | 5
      mask TypeOptions isrPriority: 0 | 1 | 2 | 3 | 4 | 5 | 6 | 7 | 8 | 9 | 10 | 11 | 12 | 13 | 14 | 15
      mask Display:
      | disp(st);
      | port_label('output',1,'trigger')
  eTimer ISR enable-disable : S-Function  FunctionName=eTimer_564xl_disable_interrupt  Parameters=uint16(subMod),uint16(channel),uint16(INTDMA)  SFunctionDeploymentMode=off  EnableBusSupport=off  mask(eTimer_564xL_disable_interrupt){SubModule=0, Timerchan=0, subMod=0, channel=0, INTDMA=0, TCFIE=off, TCF1IE=off, TCF2IE=off, TOFIE=off, IELFIE=off, IEHFIE=off, ICF1IE=off, ICF2IE=off}
      mask prompts: Timerchan "Channel"; TCFIE "Enable Compare interrupt"; TCF1IE "Enable Compare 1 interrupt"; TCF2IE "Enable Compare 2 interrupt"; TOFIE "Enable Overflow interrupt"; IELFIE "Enable Input Low Edge interrupt"; IEHFIE "Ebable Input High Edge interrupt"; ICF1IE "Ebable Input Capture 1 interrupt"; ICF2IE "Ebable Input Capture 2 interrupt"
      mask help: eTimer interrupt enable/disable
      mask init:
      | SubMod = get_param(gcb,'SubModule');
      | Chan = get_param(gcb,'TimerChan');
      | 
      | set_param(gcb,'subMod',num2str(SubMod));
      | set_param(gcb,'channel',num2str(Chan));
      | 
      | INTDMA = uint16(0);
      | if strcmp(get_param(gcb,'TCFIE'),'on')==1
      |     INTDMA = bitset(uint16(INTDMA),1);
      | end
      | if strcmp(get_param(gcb,'TCF1IE'),'on')==1
      |     INTDMA = bitset(uint16(INTDMA),2);
      | end
      | if strcmp(get_param(gcb,'TCF2IE'),'on')==1
      |     INTDMA = bitset(uint16(INTDMA),3);
      | end
      | if strcmp(get_param(gcb,'TOFIE'),'on')==1
      |     INTDMA = bitset(uint16(INTDMA),4);
      | end
      | if strcmp(get_param(gcb,'IELFIE'),'on')==1
      |     INTDMA = bitset(uint16(INTDMA),5);
      | end
      | if strcmp(get_param(gcb,'IEHFIE'),'on')==1
      |     INTDMA = bitset(uint16(INTDMA),6);
      | end
      | if strcmp(get_param(gcb,'ICF1IE'),'on')==1
      |     INTDMA = bitset(uint16(INTDMA),7);
      | end
      | if strcmp(get_param(gcb,'ICF2IE'),'on')==1
      |     INTDMA = bitset(uint16(INTDMA),8);
      | end
      | set_param(gcb,'INTDMA',num2str(INTDMA));
      | 
      | crlf= sprintf('\n');
      | st=['Sub Module ',SubMod ,' Channel ',Chan,crlf,'Interrupt Enable (INTDMA): ',dec2bin(INTDMA,16)];
      mask Help: web([rappid_block_help,filesep,'eTimer_isr_enable.htm']);
      mask TypeOptions SubModule: 0 | 1 | 2
      mask TypeOptions Timerchan: 0 | 1 | 2 | 3 | 4 | 5
      mask Display: disp(st);
  eTimer capture : S-Function  FunctionName=eTimer_564xl_capture  Parameters=uint16(subMod),uint16(channel)  SFunctionDeploymentMode=off  EnableBusSupport=off  mask(eTimer_564xL_capture){SubModule=0, Timerchan=0, subMod=0, channel=0}
      mask prompts: Timerchan "Channel"
      mask help: eTimer capture values
      mask init:
      | SubMod = get_param(gcb,'SubModule');
      | Chan = get_param(gcb,'TimerChan');
      | 
      | set_param(gcb,'subMod',num2str(SubMod));
      | set_param(gcb,'channel',num2str(Chan));
      | crlf= sprintf('\n');
      | st=['Sub Module ',SubMod ,' Channel ',Chan];
      mask Help: web([rappid_block_help,filesep,'eTimer_capture.htm']);
      mask TypeOptions SubModule: 0 | 1 | 2
      mask TypeOptions Timerchan: 0 | 1 | 2 | 3 | 4 | 5
      mask Display:
      | disp(st);
      | port_label('output',1,'CAPT1 FIFO length');
      | port_label('output',2,'CAPT1 FIFO');
      | port_label('output',3,'CAPT2 FIFO length');
      | port_label('output',4,'CAPT2 FIFO');
  eTimer configuration : S-Function  FunctionName=eTimer_564xL_config  Parameters=uint16(subMod),uint16(channel),uint16(pcrNum0),uint16(pcrNum1),uint16(pcrNum2),uint16(pcrNum3),uint16(pcrNum4),uint16(pcrNum5),uint16(CNTMODE),uint16(OUTMODE),uint16(ONCE),uint16(LENGTH),uint16(DIR),uint16(OEN),uint16(COINIT),uint16(STPEN),uint16(ROC),uint16(PRISRC),uint16(SECSRC),uint16(PIPS),uint16(SIPS),uint16(OPS),uint16(MSTR),uint16(VAL),uint16(COFRC),uint16(CLC1),uint16(CLC2),uint16(CMPMODE),uint16(CPT1MODE),uint16(CPT2MODE),uint16(ONESHOT),uint16(CFWM),uint16(CNTRinit),uint16(COMP1init),uint16(COMP2init),uint16(FILT),uint16(INTDMA)  SFunctionDeploymentMode=off  EnableBusSupport=off  mask(eTimer_564xL_config){SubModule=0, TimerChan=0, subMod=0, channel=0, CountMode=000 - No Operation, CNTMODE=0, CountOnce=0 - Count repeatedly, ONCE=0, CountLength=0 - Continue counting to roll over, LENGTH=0, CountDirection=0 - Count up, DIR=0, OutputEnable=0 - The external pin is configured as an input, OEN=0, CoChanInit=00 - Other channels cannot force re-initialization of this channel, COINIT=0, StopAction=0 - Output enable is unaffected by stop mode, STPEN=0, ReloadOnCapt=00 - Do not reload the counter on a capture event, ROC=0, PrimarySource=00000 - Counter #0 input pin, PRISRC=0, PrimSrcPol=0 - True polarity, PIPS=0, SecondarySource=00000 - Counter #0 input pin, SECSRC=0, SecSrcPol=0 - True polarity, SIPS=0, FILT_CNT=0, FILT_PER=0, FILT=0, OutputMode=0000 - Software controlled, OUTMODE=0, OutputPol=0 - True polarity, OPS=0, MasterMode=0 - Disable broadcast of this channel output, MSTR=0, ForcedOutVal=0, VAL=0, CoForce=0 - Other channels cannot force this channel output, COFRC=0, CompLoad1=000 - COMP1 is never preload, CLC1=0, CompLoad2=000 - COMP2 is never preload, CLC2=0, CompareMode=00 - COMP1 and COMP2  are used when the counter is counting up, CMPMODE=0, CaptMode1=00 - Capture disabled, CPT1MODE=0, CaptMode2=00 - Capture disabled, CPT2MODE=0, OneShCaptMode=0 - Free running mode is selected, ONESHOT=0, CaptFIFO=0, CFWM=0, CNTRinit=0, COMP1init=0, COMP2init=0, mod0ch0pin=None, mod0ch1pin=None, mod0ch2pin=None, mod0ch3pin=None, mod0ch4pin=None, mod0ch5pin=None, mod1ch0pin=None, mod1ch1pin=None, mod1ch2pin=None, mod1ch3pin=None, mod1ch4pin=None, mod1ch5pin=None, mod2ch0pin=None, mod2ch1pin=None, mod2ch2pin=None, mod2ch3pin=None, mod2ch4pin=None, mod2ch5pin=None, pcrNum0=255, pcrNum1=255, pcrNum2=255, pcrNum3=255, pcrNum4=255, pcrNum5=255, TCFIE=off, TCF1IE=off, TCF2IE=off, TOFIE=off, IELFIE=off, IEHFIE=off, ICF1IE=off, ICF2IE=off, INTDMA=0}
      mask prompts: TimerChan "Channel"; CountMode "Count mode"; CountOnce "Count once"; CountLength "Count length"; CountDirection "Count Direction"; OutputEnable "Output Enable"; CoChanInit "Co-channel initialization"; StopAction "Stop Action"; ReloadOnCapt "Reload on Capture"; PrimarySource "Primary count source"; PrimSrcPol "Primary source polarity"; SecondarySource "Secondary count source"; SecSrcPol "Secondary source polarity"; FILT_CNT "Input Filter Sample Count (0..7)"; FILT_PER "Input Filter Sample Period (0..255)"; OutputMode "Output mode"; OutputPol "Output polarity"; MasterMode "Master mode"; ForcedOutVal "Forced output value"; CoForce "Co-channel output force"; CompLoad1 "Compare Load 1"; CompLoad2 "Compare Load  2"; CompareMode "Compare Mode"; CaptMode1 "Capture 1 Mode"; CaptMode2 "Capture 2 Mode"; OneShCaptMode "One Shot Capture Mode"; CaptFIFO "Capture FIFO water mark"; CNTRinit "Counter initialization value"; COMP1init "Comparator 1 initialization value"; COMP2init "Comparator 2 initialization value"; mod0ch0pin "eTimer #0 Counter #0 pin"; mod0ch1pin "eTimer #0 Counter #1 pin"; mod0ch2pin "eTimer #0 Counter #2 pin"; mod0ch3pin "eTimer #0 Counter #3 pin"; mod0ch4pin "eTimer #0 Counter #4 pin"; mod0ch5pin "eTimer #0 Counter #5 pin"; mod1ch0pin "eTimer #1 Counter #0 pin"; mod1ch1pin "eTimer #1 Counter #1 pin"; mod1ch2pin "eTimer #1 Counter #2 pin"; mod1ch3pin "eTimer #1 Counter #3 pin"; mod1ch4pin "eTimer #1 Counter #4 pin"; mod1ch5pin "eTimer #1 Counter #5 pin"; mod2ch0pin "eTimer #2 Counter #0 pin"; mod2ch1pin "eTimer #2 Counter #1 pin"; mod2ch2pin "eTimer #2 Counter #2 pin"; mod2ch3pin "eTimer #2 Counter #3 pin"; mod2ch4pin "eTimer #2 Counter #4 pin"; mod2ch5pin "eTimer #2 Counter #5 pin"; TCFIE "Compare interrupt"; TCF1IE "Compare 1 interrupt"; TCF2IE "Compare 2 interrupt"; TOFIE "Overflow interrupt"; IELFIE "Input Low Edge interrupt"; IEHFIE "Input High Edge interrupt"; ICF1IE "Input Capture 1 interrupt"; ICF2IE "Input Capture 2 interrupt"
      mask help: eTimer configuration
      mask init:
      | SubMod = get_param(gcb,'SubModule');
      | Chan = get_param(gcb,'TimerChan');
      | CountMode = get_param(gcb,'CountMode');
      | OutputMode = get_param(gcb,'OutputMode');
      | CountOnce = get_param(gcb,'CountOnce');
      | CountLength = get_param(gcb,'CountLength');
      | CountDirection = get_param(gcb,'CountDirection');
      | OutputEnable = get_param(gcb,'OutputEnable');
      | CoChanInit = get_param(gcb,'CoChanInit');
      | StopAction = get_param(gcb,'StopAction');
      | ReloadOnCapt = get_param(gcb,'ReloadOnCapt');
      | PrimarySource = get_param(gcb,'PrimarySource');
      | SecondarySource = get_param(gcb,'SecondarySource');
      | PrimSrcPol = get_param(gcb,'PrimSrcPol');
      | SecSrcPol = get_param(gcb,'SecSrcPol');
      | OutputPol = get_param(gcb,'OutputPol');
      | MasterMode = get_param(gcb,'MasterMode');
      | ForcedOutVal = get_param(gcb,'ForcedOutVal');
      | CoForce = get_param(gcb,'CoForce');
      | CompLoad1 = get_param(gcb,'CompLoad1');
      | CompLoad2 = get_param(gcb,'CompLoad2');
      | CompareMode = get_param(gcb,'CompareMode');
      | CaptMode1 = get_param(gcb,'CaptMode1');
      | CaptMode2 = get_param(gcb,'CaptMode2');
      | OneShCaptMode = get_param(gcb,'OneShCaptMode');
      | CaptFIFO = get_param(gcb,'CaptFIFO');
      | 
      | set_param(gcb,'subMod',num2str(SubMod));
      | set_param(gcb,'channel',num2str(Chan));
      | set_param(gcb,'CNTMODE',num2str(bin2dec(CountMode(1:3))));
      | set_param(gcb,'OUTMODE',num2str(bin2dec(OutputMode(1:4))));
      | set_param(gcb,'ONCE',num2str(bin2dec(CountOnce(1:1))));
      | set_param(gcb,'LENGTH',num2str(bin2dec(CountLength(1:1))));
      | set_param(gcb,'DIR',num2str(bin2dec(CountDirection(1:1))));
      | set_param(gcb,'OEN',num2str(bin2dec(OutputEnable(1:1))));
      | set_param(gcb,'COINIT',num2str(bin2dec(CoChanInit(1:2))));
      | set_param(gcb,'STPEN',num2str(bin2dec(StopAction(1:1))));
      | set_param(gcb,'ROC',num2str(bin2dec(ReloadOnCapt(1:2))));
      | set_param(gcb,'PRISRC',num2str(bin2dec(PrimarySource(1:5))));
      | set_param(gcb,'SECSRC',num2str(bin2dec(SecondarySource(1:5))));
      | set_param(gcb,'PIPS',num2str(bin2dec(PrimSrcPol(1:1))));
      | set_param(gcb,'SIPS',num2str(bin2dec(SecSrcPol(1:1))));
      | set_param(gcb,'OPS',num2str(bin2dec(OutputPol(1:1))));
      | set_param(gcb,'MSTR',num2str(bin2dec(MasterMode(1:1))));
      | set_param(gcb,'VAL',num2str(bin2dec(ForcedOutVal(1:1))));
      | set_param(gcb,'COFRC',num2str(bin2dec(CoForce(1:1))));
      | set_param(gcb,'CLC1',num2str(bin2dec(CompLoad1(1:3))));
      | set_param(gcb,'CLC2',num2str(bin2dec(CompLoad2(1:3))));
      | set_param(gcb,'CMPMODE',num2str(bin2dec(CompareMode(1:2))));
      | set_param(gcb,'CPT1MODE',num2str(bin2dec(CaptMode1(1:2))));
      | set_param(gcb,'CPT2MODE',num2str(bin2dec(CaptMode2(1:2))));
      | set_param(gcb,'ONESHOT',num2str(bin2dec(OneShCaptMode(1:1))));
      | set_param(gcb,'CFWM',num2str(CaptFIFO));
      | 
      | for i = 0:5
      |    pcrStr = get_param(gcb,['mod',SubMod,'ch',num2str(i),'pin']);
      |    if strcmp(pcrStr,'None')==1
      |       set_param(gcb,['pcrNum',num2str(i)],'255');
      |    else    
      |       posColon = findstr(pcrStr, ':');
      |       num = strtrim(pcrStr(1:posColon(1)-1));
      |       set_param(gcb,['pcrNum',num2str(i)],num);
      |    end
      | end
      | 
      | FiltCnt = bitand(uint16(str2num(get_param(gcb,'FILT_CNT'))),7);
      | FiltPer = bitand(uint16(str2num(get_param(gcb,'FILT_PER'))),255);
      | Filter = bitor(bitshift(FiltCnt,8),FiltPer);
      | set_param(gcb,'FILT',num2str(Filter));
      | 
      | INTDMA = uint16(0);
      | if strcmp(get_param(gcb,'TCFIE'),'on')==1
      |     INTDMA = bitset(uint16(INTDMA),1);
      | end
      | if strcmp(get_param(gcb,'TCF1IE'),'on')==1
      |     INTDMA = bitset(uint16(INTDMA),2);
      | end
      | if strcmp(get_param(gcb,'TCF2IE'),'on')==1
      |     INTDMA = bitset(uint16(INTDMA),3);
      | end
      | if strcmp(get_param(gcb,'TOFIE'),'on')==1
      |     INTDMA = bitset(uint16(INTDMA),4);
      | end
      | if strcmp(get_param(gcb,'IELFIE'),'on')==1
      |     INTDMA = bitset(uint16(INTDMA),5);
      | end
      | if strcmp(get_param(gcb,'IEHFIE'),'on')==1
      |     INTDMA = bitset(uint16(INTDMA),6);
      | end
      | if strcmp(get_param(gcb,'ICF1IE'),'on')==1
      |     INTDMA = bitset(uint16(INTDMA),7);
      | end
      | if strcmp(get_param(gcb,'ICF2IE'),'on')==1
      |     INTDMA = bitset(uint16(INTDMA),8);
      | end
      | set_param(gcb,'INTDMA',num2str(INTDMA));
      | 
      | crlf= sprintf('\n');
      | st=['Sub Module ',SubMod ,' Channel ',Chan,crlf,'Count mode: ',CountMode,crlf,...
      |     'Output mode: ',OutputMode,crlf,'PrimarySource: ',PrimarySource,crlf,...
      |     'SecondarySource: ',SecondarySource];
      mask Help: web([rappid_block_help,filesep,'eTimer_config.htm']);
      mask TypeOptions SubModule: 0 | 1 | 2
      mask Callback SubModule:
      | subMod = str2num(get_param(gcb,'SubModule'));
      | channel = str2num(get_param(gcb,'TimerChan'));
      | index1 = subMod * 6;
      | index2 = subMod * 6 + 5;
      | 
      | MaskVisibilities = get_param(gcb,'MaskVisibilities');
      | for i = 0:17
      |     if (i < index1)
      |         MaskVisibilities{59+i} = 'off';
      |     elseif (i > index2)
      |         MaskVisibilities{59+i} = 'off';
      |     else
      |         MaskVisibilities{59+i} = 'on';
      |     end
      | end
      | set_param(gcb,'MaskVisibilities',MaskVisibilities);
      mask TypeOptions TimerChan: 0 | 1 | 2 | 3 | 4 | 5
      mask TypeOptions CountMode: 000 - No Operation | 001 - Count rising edges of primary source | 010 - Count rising and falling edges of primary source | 011 - Count rising edges of primary source while secondary input high active | 100 - Quadrature count mode using primary and secondary sources | 101 - Count primary source rising edges while secondary source specifies direction | 110 - Edge of secondary source triggers primary count till compare | 111 - Cascaded counter mode
      mask TypeOptions CountOnce: 0 - Count repeatedly | 1 - Count until compare and then stop
      mask TypeOptions CountLength: 0 - Continue counting to roll over | 1 - Count until compare and then reinitialize
      mask TypeOptions CountDirection: 0 - Count up | 1 - Count down
      mask TypeOptions OutputEnable: 0 - The external pin is configured as an input | 1 - Output signal is driven to the external pin
      mask TypeOptions CoChanInit: 00 - Other channels cannot force re-initialization of this channel | 01 - Other channels may force re-initialization of channel counter with LOAD | 10 - Other channels may force re-initialization of channel counter with CMPLD1 or CMPLD2
      mask TypeOptions StopAction: 0 - Output enable is unaffected by stop mode | 1 - Output enable is disabled during stop mode
      mask TypeOptions ReloadOnCapt: 00 - Do not reload the counter on a capture event | 01 - Reload the counter on a capture 1 event | 10 - Reload the counter on a capture 2 event | 11 - Reload the counter on both a capture 1 event and a capture 2 event
      mask TypeOptions PrimarySource: 00000 - Counter #0 input pin | 00001 - Counter #1 input pin | 00010 - Counter #2 input pin | 00011 - Counter #3 input pin | 00100 - Counter #4 input pin | 00101 - Counter #5 input pin | 01000 - Auxiliary input #0 pin | 01001 - Auxiliary input #1 pin | 01010 - Auxiliary input #2 pin | 10000 - Counter #0 output | 10001 - Counter #1 output | 10010 - Counter #2 output | 10011 - Counter #3 output | 10100 - Counter #4 output | 10101 - Counter #5 output | 11000 - IP Bus clock divide by 1 prescaler | 11001 - IP Bus clock divide by 2 prescaler | 11010 - IP Bus clock divide by 4 prescaler | 11011 - IP Bus clock divide by 8 prescaler | 11100 - IP Bus clock divide by 16 prescaler | 11101 - IP Bus clock divide by 32 prescaler | 11110 - IP Bus clock divide by 64 prescaler | 11111 - IP Bus clock divide by 128 prescaler
      mask TypeOptions PrimSrcPol: 0 - True polarity | 1 - Inverted polarity
      mask TypeOptions SecondarySource: 00000 - Counter #0 input pin | 00001 - Counter #1 input pin | 00010 - Counter #2 input pin | 00011 - Counter #3 input pin | 00100 - Counter #4 input pin | 00101 - Counter #5 input pin | 01000 - Auxiliary input #0 pin | 01001 - Auxiliary input #1 pin | 01010 - Auxiliary input #2 pin | 10000 - Counter #0 output | 10001 - Counter #1 output | 10010 - Counter #2 output | 10011 - Counter #3 output | 10100 - Counter #4 output | 10101 - Counter #5 output
      mask TypeOptions SecSrcPol: 0 - True polarity | 1 - Inverted polarity
      mask TypeOptions OutputMode: 0000 - Software controlled | 0001 - Clear output on successful compare (COMP1 or COMP2) | 0010 - Set  output on successful compare (COMP1 or COMP2) | 0011 - Toggle output on successful compare (COMP1 or COMP2) | 0100 - Toggle output using alternating compare registers | 0101 - Set output on compare with COMP1 and clear on secondary source input edge | 0110 - Set output on compare with COMP2 and clear on secondary source input edge | 0111 - Set output on compare and clear on counter roll-over | 1000 - Set output on compare on COMP1 and clear on compare on COMP2 | 1001 - Asserted while counter is active and cleared when counter is stopped | 1010 - Asserted when counting up and cleared when counting down | 1111 - Enable gated clock output while counter is active
      mask TypeOptions OutputPol: 0 - True polarity | 1 - Inverted polarity
      mask TypeOptions MasterMode: 0 - Disable broadcast of this channel output | 1 - Enable broadcast of this channel output
      mask TypeOptions ForcedOutVal: 0 | 1
      mask TypeOptions CoForce: 0 - Other channels cannot force this channel output | 1 - Other channels may force this channel output
      mask TypeOptions CompLoad1: 000 - COMP1 is never preload | 010 - Load COMP1 with CMPLD1 upon successful compare with the value in COMP1 | 011 - Load COMP1 with CMPLD1 upon successful compare with the value in COMP2 | 100 - Load COMP1 with CMPLD2 upon successful compare with the value in COMP1 | 101 - Load COMP1 with CMPLD2 upon successful compare with the value in COMP2 | 110 - Load CNTR with CMPLD1 upon successful compare with the value in COMP1 | 111 - Load CNTR with CMPLD1 upon successful compare with the value in COMP2
      mask TypeOptions CompLoad2: 000 - COMP2 is never preload | 010 - Load COMP2 with CMPLD1 upon successful compare with the value in COMP1 | 011 - Load COMP2 with CMPLD1 upon successful compare with the value in COMP2 | 100 - Load COMP2 with CMPLD2 upon successful compare with the value in COMP1 | 101 - Load COMP2 with CMPLD2 upon successful compare with the value in COMP2 | 110 - Load CNTR with CMPLD2 upon successful compare with the value in COMP1 | 111 - Load CNTR with CMPLD2 upon successful compare with the value in COMP2
      mask TypeOptions CompareMode: 00 - COMP1 and COMP2  are used when the counter is counting up | 01 - COMP1  is used when the counter is counting down and COMP2 when counting up | 10 - COMP1  is used when the counter is counting up and COMP2 when counting down | 11 - COMP1 and COMP2  are used when the counter is counting down
      mask TypeOptions CaptMode1: 00 - Capture disabled | 01 - Capture falling edges | 10 - Capture rising edges | 11 - Capture any edge
      mask TypeOptions CaptMode2: 00 - Capture disabled | 01 - Capture falling edges | 10 - Capture rising edges | 11 - Capture any edge
      mask TypeOptions OneShCaptMode: 0 - Free running mode is selected | 1 - One shot mode is selected
      mask TypeOptions CaptFIFO: 0 | 1 | 2 | 3
      mask TypeOptions mod0ch0pin: None | 0   : PA0  : [ 73 ] : [ T14 ]  input/output | 58  : PD10 : [ 76 ] : [ T15 ]  input
      mask TypeOptions mod0ch1pin: None | 1   : PA1  : [ 74 ] : [ R14 ]  input/output | 59  : PD11 : [ 78 ] : [ R16 ]  input
      mask TypeOptions mod0ch2pin: None | 2   : PA2  : [ 84 ] : [ N16 ]  input/output | 80  : PF0  : [ 133 ] : [ D7 ]  input
      mask TypeOptions mod0ch3pin: None | 3   : PA3  : [ 92 ] : [ K17 ]  input/output | 62  : PD14 : [ 105 ] : [ D16 ]  input
      mask TypeOptions mod0ch4pin: None | 4   : PA4  : [ 108 ] : [ C16 ]  input/output | 30  : PB14 : [ 64 ] : [ P11 ]  input | 43  : PC11 : [ 80 ] : [ M14 ]  input/output | 99  : PG3  : [ 104 ] : [ D17 ]  input
      mask TypeOptions mod0ch5pin: None | 24  : PB8  : [ 47 ] : [ P7 ]  input | 44  : PC12 : [ 82 ] : [ N15 ]  input/output | 77  : PE13 : [ 117 ] : [ D12 ]  input/output | 100 : PG4  : [ 100 ] : [ F17 ]  input
      mask TypeOptions mod1ch0pin: None | 4   : PA4  : [ 108 ] : [ C16 ]  input/output | 47  : PC15 : [ 124 ] : [ A8 ]  input/output
      mask TypeOptions mod1ch1pin: None | 45  : PC13 : [ 101 ] : [ F15 ]  input/output | 48  : PD0  : [ 125 ] : [ B8 ]  input/output
      mask TypeOptions mod1ch2pin: None | 16  : PB0  : [ 109 ] : [ B15 ]  input/output | 46  : PC14 : [ 103 ] : [ E15 ]  input/output | 49  : PD1  : [ 3 ] : [ E3 ]  input/output
      mask TypeOptions mod1ch3pin: None | 17  : PB1  : [ 110 ] : [ C14 ]  input/output | 50  : PD2  : [ 140 ] : [ C5 ]  input/output | 92  : PF12 : [ 106 ] : [ C17 ]  input/output
      mask TypeOptions mod1ch4pin: None | 14  : PA14 : [ 143 ] : [ B4 ]  input/output | 51  : PD3  : [ 128 ] : [ A7 ]  input/output | 56  : PD8  : [ 32 ] : [ M3 ]  input/output | 93  : PF13 : [ 112 ] : [ B14 ]  input/output
      mask TypeOptions mod1ch5pin: None | 5   : PA5  : [ 14 ] : [ H4 ]  input/output | 15  : PA15 : [ 144 ] : [ D3 ]  input/output | 52  : PD4  : [ 129 ] : [ B7 ]  input/output | 78  : PE14 : [ 119 ] : [ B12 ]  input/output
      mask TypeOptions mod2ch0pin: None | 116 : PH4  : [ --- ] : [ L16 ]  input/output | 128 : PI0  : [ --- ] : [ C9 ]  input/output
      mask TypeOptions mod2ch1pin: None | 119 : PH7  : [ --- ] : [ K16 ]  input/output | 129 : PI1  : [ --- ] : [ C12 ]  input/output
      mask TypeOptions mod2ch2pin: None | 122 : PH10 : [ --- ] : [ A11 ]  input/output | 130 : PI2  : [ --- ] : [ F16 ]  input/output
      mask TypeOptions mod2ch3pin: None | 125 : PH13 : [ --- ] : [ G15 ]  input/output | 131 : PI3  : [ --- ] : [ E17 ]  input/output
      mask TypeOptions mod2ch4pin: None | 126 : PH14 : [ --- ] : [ A12 ]  input/output
      mask TypeOptions mod2ch5pin: None | 127 : PH15 : [ --- ] : [ J17 ]  input/output
      mask Display: disp(st);
  eTimer pre-load : S-Function  FunctionName=eTimer_564xl_preload  Parameters=uint16(subMod),uint16(channel)  SFunctionDeploymentMode=off  EnableBusSupport=off  mask(eTimer_564xL_preload){SubModule=0, Timerchan=0, subMod=0, channel=0}
      mask prompts: Timerchan "Channel"
      mask help: eTimer counter and comparator pre-loading
      mask init: same as rappid_564xl_ec_toolbox/MPC564xL/Motor Control Blocks/eTimer capture
